simulink model "Channelizer"  (R2023a)
settings: Solver=VariableStepAuto  StartTime=0.0  StopTime=inf  RelTol=1e-3
InitFcn:
  | init;
values from neighbouring files (symbols this model uses):
  ch0_en = 0    [init.m]
  ch0_qam = 0    [init.m]
  ch0_swp = 0    [init.m]
  ch10_en = 0    [init.m]
  ch10_qam = 0    [init.m]
  ch10_swp = 0    [init.m]
  ch11_en = 0    [init.m]
  ch11_qam = 0    [init.m]
  ch11_swp = 0    [init.m]
  ch12_en = 0    [init.m]
  ch12_qam = 0    [init.m]
  ch12_swp = 0    [init.m]
  ch13_en = 0    [init.m]
  ch13_qam = 0    [init.m]
  ch13_swp = 0    [init.m]
  ch14_en = 0    [init.m]
  ch14_qam = 0    [init.m]
  ch14_swp = 0    [init.m]
  ch15_en = 0    [init.m]
  ch15_qam = 0    [init.m]
  ch15_swp = 0    [init.m]
  ch1_en = 1    [init.m]
  ch1_qam = 0    [init.m]
  ch1_swp = 0    [init.m]
  ch2_en = 1    [init.m]
  ch2_qam = 0    [init.m]
  ch2_swp = 0    [init.m]
  ch3_en = 0    [init.m]
  ch3_qam = 0    [init.m]
  ch3_swp = 0    [init.m]
  ch4_en = 0    [init.m]
  ch4_qam = 0    [init.m]
  ch4_swp = 0    [init.m]
  ch5_en = 1    [init.m]
  ch5_qam = 1    [init.m]
  ch5_swp = 0    [init.m]
  ch6_en = 1    [init.m]
  ch6_qam = 1    [init.m]
  ch6_swp = 0    [init.m]
  ch7_en = 0    [init.m]
  ch7_qam = 0    [init.m]
  ch7_swp = 0    [init.m]
  ch8_en = 0    [init.m]
  ch8_qam = 0    [init.m]
  ch8_swp = 0    [init.m]
  ch9_en = 0    [init.m]
  ch9_qam = 0    [init.m]
  ch9_swp = 0    [init.m]
  ch_filt_coef = 28 * ch_filt_coef / sum(ch_filt_coef(:))    [init.m]
  N = 512    [init.m]
  spec1_ch = 1    [init.m]
  spec2_ch = 2    [init.m]
  spec3_ch = 5    [init.m]
  spec4_ch = 6    [init.m]
  swp_rate0 = 0    [init.m]
  swp_rate1 = 0    [init.m]
  swp_rate10 = 0    [init.m]
  swp_rate11 = 0    [init.m]
  swp_rate12 = 0    [init.m]
  swp_rate13 = 0    [init.m]
  swp_rate14 = 0    [init.m]
  swp_rate15 = 0    [init.m]
  swp_rate2 = 0    [init.m]
  swp_rate3 = 0    [init.m]
  swp_rate4 = 0    [init.m]
  swp_rate5 = 0    [init.m]
  swp_rate6 = 0    [init.m]
  swp_rate7 = 0    [init.m]
  swp_rate8 = 0    [init.m]
  swp_rate9 = 0    [init.m]
  Ts = 16*(7/4)/8.75e9    (= 3.2e-09)    [init.m]
undefined symbols (not defined in the file or in its folder): S, vsva2197, xcvc1902
libraries: aieBasic x56, aieUtilities x47, dspswit3 x16, dspsigops x16, hlsBasic x3, dspindex x1, vmcUtilities x1, commchan3 x1
(part 3 of 4)

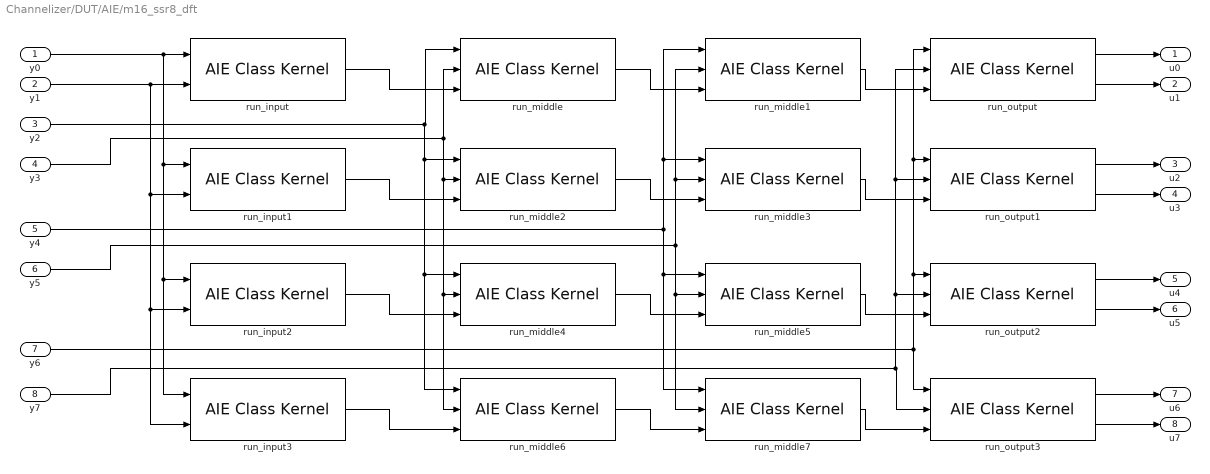
== system Channelizer/DUT/AIE/m16_ssr8_dft ==
  y0 : Inport
  y1 : Inport  Port=2
  y2 : Inport  Port=3
  y3 : Inport  Port=4
  y4 : Inport  Port=5
  y5 : Inport  Port=6
  y6 : Inport  Port=7
  y7 : Inport  Port=8
  run_input : aieBasic/AIE Class Kernel  KernelAllAttrs=|  PortNames={'sig0_i'; 'sig1_i'; 'acc_o'}  PortSerializedTypes={'{Q2{P{Tinput_stream{1{t{ETT_DATA}}}}}}'; '{Q2{P{Tinput_stream{1{t{ETT_DATA}}}}}}'; '{Q2{P{Toutput_stream{1{t{ETT_ACC}}}}}}'}  PortWindowSizes={0.000000000000000000e+00; 0.000000000000000000e+00; 0.000000000000000000e+00}  PortWindowMargins={0.000000000000000000e+00; 0.000000000000000000e+00; 0.000000000000000000e+00}  PortSynchronicities={'auto', 'auto', 'auto'}  PortSignalSizes={0.000000000000000000e+00; 0.000000000000000000e+00; 4.096000000000000000e+03}  ClassTemplateSpecKind=implicit  ClassTemplateParamNames={'TT_DATA'; 'TT_COEFF'; 'TT_ACC'; 'NSAMP'}  ClassTemplateParamKinds={'type'; 'type'; 'type'; 'nontype'}  ClassTemplateParamTypes={'typename'; 'typename'; 'typename'; 'unsigned int'}  ClassTemplateParamValues={'cint16', 'cint16', 'cacc48', '2048'}  ClassCtorParamNames={'coeff0_i'; 'coeff1_i'}  ClassCtorParamSerializedTypes={'{R{C{ETT_COEFF}8}}'; '{R{C{ETT_COEFF}8}}'}  ClassCtorParamValues={'[32767 32767 32767 32767 32767 30274+12540i 23170+23170i 12540+30274i]', '[32767 23170+23170i 0+32767i -23170+23170i 32767 12540+30274i -23170+23170i -30274-12540i]'}  ClassIndex=1  ClassCtorIndex=1  ClassTabVisible=on  ClassTemplateParamsVisible=on  ClassCtorDeclVisible=on  ClassCtorParamsVisible=on  FunctionTabVisible=on  FunctionDecl=|  PortAttrs={ 'input', 'sig0_i', 'input_stream< TT_DATA > * restrict', '', '', '', ''; 'input', 'sig1_i', 'input_stream< TT_DATA > * restrict', '', '', '', ''; 'output', 'acc_o', 'output_stream< TT_ACC > * restrict', '', '', '', '8*N' }  PortAttrsEnables={'off', 'off', 'off', 'off', 'off', 'off', 'off';'off', 'off', 'off', 'off', 'off', 'off', 'off';'off', 'off', 'off', 'off', 'off', 'off', 'on'}  SampleTime=-1  ClassDeclTypeOptions=C[1 1]@t106@template < typename TT_DATA, typename TT_COEFF, typename TT_ACC, unsigned int NSAMP > class dft_1xN_input;  ClassDecl=template < typename TT_DATA, typename TT_COEFF, typename TT_ACC, unsigned int NSAMP > class dft_1xN_input;  ClassTemplateParams={ 'TT_DATA', 'typename', 'cint16'; 'TT_COEFF', 'typename', 'cint16'; 'TT_ACC', 'typename', 'cacc48'; 'NSAMP', 'unsigned int', '4*N' }  ClassTemplateParamsEnables={'off', 'off', 'on';'off', 'off', 'on';'off', 'off', 'on';'off', 'off', 'on'}  ClassCtorDeclTypeOptions=C[1 1]@t75@dft_1xN_input(TT_COEFF ( & coeff0_i ) [ 8 ], TT_COEFF ( & coeff1_i ) [ 8 ])  ClassCtorDecl=dft_1xN_input(TT_COEFF ( & coeff0_i ) [ 8 ], TT_COEFF ( & coeff1_i ) [ 8 ])  ClassCtorParams={ 'coeff0_i', 'TT_COEFF ( &) [ 8 ]', 'twidA0(1,:)'; 'coeff1_i', 'TT_COEFF ( &) [ 8 ]', 'twidA1(1,:)' }  KernelHeaderFile=aie/dft_1xN_widget.h  KernelClassName=dft_1xN_input  KernelFunction=run_input  KernelSourceFile=aie/dft_1xN_widget.cpp  KernelSearchPaths={}  PreProcOptions={}  blockJsonConstraints=[]
      KernelAllAttrs=|
      | s[12;12;9;9;19;14;21;23;21;23;24;21;15;17;12;24;26;26;26;27;28;9;21;23;23;23;24;25;14;19;19;29]@FunctionNameDeclFileNamePortNamesPortTypesPortSerializedTypesPortDirectionsPortWindowSizeEnablesPortWindowMarginEnablesPortBufferSizeEnablesPortBufferMarginEnablesPortSynchronicityEnablesPortSignalSizeEnablesPortBufferSizesPortBufferMarginsFunctionDeclFunctionTemplateSpecKindFunctionTemplateParamNamesFunctionTemplateParamKindsFunctionTemplateParamTypesFunctionTemplateParamValuesFunctionTemplateParamEnablesClassDeclClassTemplateSpecKindClassTemplateParamNamesClassTemplateParamKindsClassTemplateParamTypesClassTemplateParamValuesClassTemplateParamEnablesClassCtorDeclsClassCtorParamNamesClassCtorParamTypesClassCtorParamSerializedTypes[1 1]@C[32 1]@t9@run_inputt22@../../dft_1xN_widget.hC[3 1]@t6@sig0_it6@sig1_it5@acc_oC[3 1]@t34@input_stream< TT_DATA > * restrictt34@input_stream< TT_DATA > * restrictt34@output_stream< TT_ACC > * restrictC[3 1]@t38@{Q2{P{Tinput_stream{1{t{ETT_DATA}}}}}}t38@{Q2{P{Tinput_stream{1{t{ETT_DATA}}}}}}t38@{Q2{P{Toutput_stream{1{t{ETT_ACC}}}}}}C[3 1]@t5@inputt5@inputt6@outputC[3 1]@l0@l0@l0@C[3 1]@l0@l0@l0@C[3 1]@l0@l0@l0@C[3 1]@l0@l0@l0@C[3 1]@l0@l0@l0@C[3 1]@l0@l0@l1@C[3 1]@nnnC[3 1]@nnnt245@template < typename TT_DATA, typename TT_COEFF, typename TT_ACC, unsigned int NSAMP > 
      | void dft_1xN_input::
      | run_input(input_stream< TT_DATA > * restrict sig0_i, input_stream< TT_DATA > * restrict sig1_i, output_stream< TT_ACC > * restrict acc_o)t4@nonee[0 1]@e[0 1]@e[0 1]@e[0 1]@e[0 1]@t106@template < typename TT_DATA, typename TT_COEFF, typename TT_ACC, unsigned int NSAMP > class dft_1xN_input;t8@implicitC[4 1]@t7@TT_DATAt8@TT_COEFFt6@TT_ACCt5@NSAMPC[4 1]@t4@typet4@typet4@typet7@nontypeC[4 1]@t8@typenamet8@typenamet8@typenamet12@unsigned intC[4 1]@nnnnC[4 1]@l1@l1@l1@l1@C[1 1]@t75@dft_1xN_input(TT_COEFF ( & coeff0_i ) [ 8 ], TT_COEFF ( & coeff1_i ) [ 8 ])C[1 1]@C[2 1]@t8@coeff0_it8@coeff1_iC[1 1]@C[2 1]@t19@TT_COEFF ( &) [ 8 ]t19@TT_COEFF ( &) [ 8 ]C[1 1]@C[2 1]@t18@{R{C{ETT_COEFF}8}}t18@{R{C{ETT_COEFF}8}}
      FunctionDecl=|
      | template < typename TT_DATA, typename TT_COEFF, typename TT_ACC, unsigned int NSAMP > 
      | void dft_1xN_input::
      | run_input(input_stream< TT_DATA > * restrict sig0_i, input_stream< TT_DATA > * restrict sig1_i, output_stream< TT_ACC > * restrict acc_o)
  run_input1 : aieBasic/AIE Class Kernel  KernelAllAttrs=|  PortNames={'sig0_i'; 'sig1_i'; 'acc_o'}  PortSerializedTypes={'{Q2{P{Tinput_stream{1{t{ETT_DATA}}}}}}'; '{Q2{P{Tinput_stream{1{t{ETT_DATA}}}}}}'; '{Q2{P{Toutput_stream{1{t{ETT_ACC}}}}}}'}  PortWindowSizes={0.000000000000000000e+00; 0.000000000000000000e+00; 0.000000000000000000e+00}  PortWindowMargins={0.000000000000000000e+00; 0.000000000000000000e+00; 0.000000000000000000e+00}  PortSynchronicities={'auto', 'auto', 'auto'}  PortSignalSizes={0.000000000000000000e+00; 0.000000000000000000e+00; 4.096000000000000000e+03}  ClassTemplateSpecKind=implicit  ClassTemplateParamNames={'TT_DATA'; 'TT_COEFF'; 'TT_ACC'; 'NSAMP'}  ClassTemplateParamKinds={'type'; 'type'; 'type'; 'nontype'}  ClassTemplateParamTypes={'typename'; 'typename'; 'typename'; 'unsigned int'}  ClassTemplateParamValues={'cint16', 'cint16', 'cacc48', '2048'}  ClassCtorParamNames={'coeff0_i'; 'coeff1_i'}  ClassCtorParamSerializedTypes={'{R{C{ETT_COEFF}8}}'; '{R{C{ETT_COEFF}8}}'}  ClassCtorParamValues={'[32767 32767 32767 32767 0+32767i -12540+30274i -23170+23170i -30274+12540i]', '[-32768 -23170-23170i 0-32768i 23170-23170i 0-32768i 30274-12540i 23170+23170i -12540+30274i]'}  ClassIndex=1  ClassCtorIndex=1  ClassTabVisible=on  ClassTemplateParamsVisible=on  ClassCtorDeclVisible=on  ClassCtorParamsVisible=on  FunctionTabVisible=on  FunctionDecl=|  PortAttrs={ 'input', 'sig0_i', 'input_stream< TT_DATA > * restrict', '', '', '', ''; 'input', 'sig1_i', 'input_stream< TT_DATA > * restrict', '', '', '', ''; 'output', 'acc_o', 'output_stream< TT_ACC > * restrict', '', '', '', '8*N' }  PortAttrsEnables={'off', 'off', 'off', 'off', 'off', 'off', 'off';'off', 'off', 'off', 'off', 'off', 'off', 'off';'off', 'off', 'off', 'off', 'off', 'off', 'on'}  SampleTime=-1  ClassDeclTypeOptions=C[1 1]@t106@template < typename TT_DATA, typename TT_COEFF, typename TT_ACC, unsigned int NSAMP > class dft_1xN_input;  ClassDecl=template < typename TT_DATA, typename TT_COEFF, typename TT_ACC, unsigned int NSAMP > class dft_1xN_input;  ClassTemplateParams={ 'TT_DATA', 'typename', 'cint16'; 'TT_COEFF', 'typename', 'cint16'; 'TT_ACC', 'typename', 'cacc48'; 'NSAMP', 'unsigned int', '4*N' }  ClassTemplateParamsEnables={'off', 'off', 'on';'off', 'off', 'on';'off', 'off', 'on';'off', 'off', 'on'}  ClassCtorDeclTypeOptions=C[1 1]@t75@dft_1xN_input(TT_COEFF ( & coeff0_i ) [ 8 ], TT_COEFF ( & coeff1_i ) [ 8 ])  ClassCtorDecl=dft_1xN_input(TT_COEFF ( & coeff0_i ) [ 8 ], TT_COEFF ( & coeff1_i ) [ 8 ])  ClassCtorParams={ 'coeff0_i', 'TT_COEFF ( &) [ 8 ]', 'twidB0(1,:)'; 'coeff1_i', 'TT_COEFF ( &) [ 8 ]', 'twidB1(1,:)' }  KernelHeaderFile=aie/dft_1xN_widget.h  KernelClassName=dft_1xN_input  KernelFunction=run_input  KernelSourceFile=aie/dft_1xN_widget.cpp  KernelSearchPaths={}  PreProcOptions={}  blockJsonConstraints=[]
      KernelAllAttrs=|
      | s[12;12;9;9;19;14;21;23;21;23;24;21;15;17;12;24;26;26;26;27;28;9;21;23;23;23;24;25;14;19;19;29]@FunctionNameDeclFileNamePortNamesPortTypesPortSerializedTypesPortDirectionsPortWindowSizeEnablesPortWindowMarginEnablesPortBufferSizeEnablesPortBufferMarginEnablesPortSynchronicityEnablesPortSignalSizeEnablesPortBufferSizesPortBufferMarginsFunctionDeclFunctionTemplateSpecKindFunctionTemplateParamNamesFunctionTemplateParamKindsFunctionTemplateParamTypesFunctionTemplateParamValuesFunctionTemplateParamEnablesClassDeclClassTemplateSpecKindClassTemplateParamNamesClassTemplateParamKindsClassTemplateParamTypesClassTemplateParamValuesClassTemplateParamEnablesClassCtorDeclsClassCtorParamNamesClassCtorParamTypesClassCtorParamSerializedTypes[1 1]@C[32 1]@t9@run_inputt22@../../dft_1xN_widget.hC[3 1]@t6@sig0_it6@sig1_it5@acc_oC[3 1]@t34@input_stream< TT_DATA > * restrictt34@input_stream< TT_DATA > * restrictt34@output_stream< TT_ACC > * restrictC[3 1]@t38@{Q2{P{Tinput_stream{1{t{ETT_DATA}}}}}}t38@{Q2{P{Tinput_stream{1{t{ETT_DATA}}}}}}t38@{Q2{P{Toutput_stream{1{t{ETT_ACC}}}}}}C[3 1]@t5@inputt5@inputt6@outputC[3 1]@l0@l0@l0@C[3 1]@l0@l0@l0@C[3 1]@l0@l0@l0@C[3 1]@l0@l0@l0@C[3 1]@l0@l0@l0@C[3 1]@l0@l0@l1@C[3 1]@nnnC[3 1]@nnnt245@template < typename TT_DATA, typename TT_COEFF, typename TT_ACC, unsigned int NSAMP > 
      | void dft_1xN_input::
      | run_input(input_stream< TT_DATA > * restrict sig0_i, input_stream< TT_DATA > * restrict sig1_i, output_stream< TT_ACC > * restrict acc_o)t4@nonee[0 1]@e[0 1]@e[0 1]@e[0 1]@e[0 1]@t106@template < typename TT_DATA, typename TT_COEFF, typename TT_ACC, unsigned int NSAMP > class dft_1xN_input;t8@implicitC[4 1]@t7@TT_DATAt8@TT_COEFFt6@TT_ACCt5@NSAMPC[4 1]@t4@typet4@typet4@typet7@nontypeC[4 1]@t8@typenamet8@typenamet8@typenamet12@unsigned intC[4 1]@nnnnC[4 1]@l1@l1@l1@l1@C[1 1]@t75@dft_1xN_input(TT_COEFF ( & coeff0_i ) [ 8 ], TT_COEFF ( & coeff1_i ) [ 8 ])C[1 1]@C[2 1]@t8@coeff0_it8@coeff1_iC[1 1]@C[2 1]@t19@TT_COEFF ( &) [ 8 ]t19@TT_COEFF ( &) [ 8 ]C[1 1]@C[2 1]@t18@{R{C{ETT_COEFF}8}}t18@{R{C{ETT_COEFF}8}}
      FunctionDecl=|
      | template < typename TT_DATA, typename TT_COEFF, typename TT_ACC, unsigned int NSAMP > 
      | void dft_1xN_input::
      | run_input(input_stream< TT_DATA > * restrict sig0_i, input_stream< TT_DATA > * restrict sig1_i, output_stream< TT_ACC > * restrict acc_o)
  run_input2 : aieBasic/AIE Class Kernel  KernelAllAttrs=|  PortNames={'sig0_i'; 'sig1_i'; 'acc_o'}  PortSerializedTypes={'{Q2{P{Tinput_stream{1{t{ETT_DATA}}}}}}'; '{Q2{P{Tinput_stream{1{t{ETT_DATA}}}}}}'; '{Q2{P{Toutput_stream{1{t{ETT_ACC}}}}}}'}  PortWindowSizes={0.000000000000000000e+00; 0.000000000000000000e+00; 0.000000000000000000e+00}  PortWindowMargins={0.000000000000000000e+00; 0.000000000000000000e+00; 0.000000000000000000e+00}  PortSynchronicities={'auto', 'auto', 'auto'}  PortSignalSizes={0.000000000000000000e+00; 0.000000000000000000e+00; 4.096000000000000000e+03}  ClassTemplateSpecKind=implicit  ClassTemplateParamNames={'TT_DATA'; 'TT_COEFF'; 'TT_ACC'; 'NSAMP'}  ClassTemplateParamKinds={'type'; 'type'; 'type'; 'nontype'}  ClassTemplateParamTypes={'typename'; 'typename'; 'typename'; 'unsigned int'}  ClassTemplateParamValues={'cint16', 'cint16', 'cacc48', '2048'}  ClassCtorParamNames={'coeff0_i'; 'coeff1_i'}  ClassCtorParamSerializedTypes={'{R{C{ETT_COEFF}8}}'; '{R{C{ETT_COEFF}8}}'}  ClassCtorParamValues={'[32767 32767 32767 32767 -32768 -30274-12540i -23170-23170i -12540-30274i]', '[32767 23170+23170i 0+32767i -23170+23170i -32768 -12540-30274i 23170-23170i 30274+12540i]'}  ClassIndex=1  ClassCtorIndex=1  ClassTabVisible=on  ClassTemplateParamsVisible=on  ClassCtorDeclVisible=on  ClassCtorParamsVisible=on  FunctionTabVisible=on  FunctionDecl=|  PortAttrs={ 'input', 'sig0_i', 'input_stream< TT_DATA > * restrict', '', '', '', ''; 'input', 'sig1_i', 'input_stream< TT_DATA > * restrict', '', '', '', ''; 'output', 'acc_o', 'output_stream< TT_ACC > * restrict', '', '', '', '8*N' }  PortAttrsEnables={'off', 'off', 'off', 'off', 'off', 'off', 'off';'off', 'off', 'off', 'off', 'off', 'off', 'off';'off', 'off', 'off', 'off', 'off', 'off', 'on'}  SampleTime=-1  ClassDeclTypeOptions=C[1 1]@t106@template < typename TT_DATA, typename TT_COEFF, typename TT_ACC, unsigned int NSAMP > class dft_1xN_input;  ClassDecl=template < typename TT_DATA, typename TT_COEFF, typename TT_ACC, unsigned int NSAMP > class dft_1xN_input;  ClassTemplateParams={ 'TT_DATA', 'typename', 'cint16'; 'TT_COEFF', 'typename', 'cint16'; 'TT_ACC', 'typename', 'cacc48'; 'NSAMP', 'unsigned int', '4*N' }  ClassTemplateParamsEnables={'off', 'off', 'on';'off', 'off', 'on';'off', 'off', 'on';'off', 'off', 'on'}  ClassCtorDeclTypeOptions=C[1 1]@t75@dft_1xN_input(TT_COEFF ( & coeff0_i ) [ 8 ], TT_COEFF ( & coeff1_i ) [ 8 ])  ClassCtorDecl=dft_1xN_input(TT_COEFF ( & coeff0_i ) [ 8 ], TT_COEFF ( & coeff1_i ) [ 8 ])  ClassCtorParams={ 'coeff0_i', 'TT_COEFF ( &) [ 8 ]', 'twidC0(1,:)'; 'coeff1_i', 'TT_COEFF ( &) [ 8 ]', 'twidC1(1,:)' }  KernelHeaderFile=aie/dft_1xN_widget.h  KernelClassName=dft_1xN_input  KernelFunction=run_input  KernelSourceFile=aie/dft_1xN_widget.cpp  KernelSearchPaths={}  PreProcOptions={}  blockJsonConstraints=[]
      KernelAllAttrs=|
      | s[12;12;9;9;19;14;21;23;21;23;24;21;15;17;12;24;26;26;26;27;28;9;21;23;23;23;24;25;14;19;19;29]@FunctionNameDeclFileNamePortNamesPortTypesPortSerializedTypesPortDirectionsPortWindowSizeEnablesPortWindowMarginEnablesPortBufferSizeEnablesPortBufferMarginEnablesPortSynchronicityEnablesPortSignalSizeEnablesPortBufferSizesPortBufferMarginsFunctionDeclFunctionTemplateSpecKindFunctionTemplateParamNamesFunctionTemplateParamKindsFunctionTemplateParamTypesFunctionTemplateParamValuesFunctionTemplateParamEnablesClassDeclClassTemplateSpecKindClassTemplateParamNamesClassTemplateParamKindsClassTemplateParamTypesClassTemplateParamValuesClassTemplateParamEnablesClassCtorDeclsClassCtorParamNamesClassCtorParamTypesClassCtorParamSerializedTypes[1 1]@C[32 1]@t9@run_inputt22@../../dft_1xN_widget.hC[3 1]@t6@sig0_it6@sig1_it5@acc_oC[3 1]@t34@input_stream< TT_DATA > * restrictt34@input_stream< TT_DATA > * restrictt34@output_stream< TT_ACC > * restrictC[3 1]@t38@{Q2{P{Tinput_stream{1{t{ETT_DATA}}}}}}t38@{Q2{P{Tinput_stream{1{t{ETT_DATA}}}}}}t38@{Q2{P{Toutput_stream{1{t{ETT_ACC}}}}}}C[3 1]@t5@inputt5@inputt6@outputC[3 1]@l0@l0@l0@C[3 1]@l0@l0@l0@C[3 1]@l0@l0@l0@C[3 1]@l0@l0@l0@C[3 1]@l0@l0@l0@C[3 1]@l0@l0@l1@C[3 1]@nnnC[3 1]@nnnt245@template < typename TT_DATA, typename TT_COEFF, typename TT_ACC, unsigned int NSAMP > 
      | void dft_1xN_input::
      | run_input(input_stream< TT_DATA > * restrict sig0_i, input_stream< TT_DATA > * restrict sig1_i, output_stream< TT_ACC > * restrict acc_o)t4@nonee[0 1]@e[0 1]@e[0 1]@e[0 1]@e[0 1]@t106@template < typename TT_DATA, typename TT_COEFF, typename TT_ACC, unsigned int NSAMP > class dft_1xN_input;t8@implicitC[4 1]@t7@TT_DATAt8@TT_COEFFt6@TT_ACCt5@NSAMPC[4 1]@t4@typet4@typet4@typet7@nontypeC[4 1]@t8@typenamet8@typenamet8@typenamet12@unsigned intC[4 1]@nnnnC[4 1]@l1@l1@l1@l1@C[1 1]@t75@dft_1xN_input(TT_COEFF ( & coeff0_i ) [ 8 ], TT_COEFF ( & coeff1_i ) [ 8 ])C[1 1]@C[2 1]@t8@coeff0_it8@coeff1_iC[1 1]@C[2 1]@t19@TT_COEFF ( &) [ 8 ]t19@TT_COEFF ( &) [ 8 ]C[1 1]@C[2 1]@t18@{R{C{ETT_COEFF}8}}t18@{R{C{ETT_COEFF}8}}
      FunctionDecl=|
      | template < typename TT_DATA, typename TT_COEFF, typename TT_ACC, unsigned int NSAMP > 
      | void dft_1xN_input::
      | run_input(input_stream< TT_DATA > * restrict sig0_i, input_stream< TT_DATA > * restrict sig1_i, output_stream< TT_ACC > * restrict acc_o)
  run_input3 : aieBasic/AIE Class Kernel  KernelAllAttrs=|  PortNames={'sig0_i'; 'sig1_i'; 'acc_o'}  PortSerializedTypes={'{Q2{P{Tinput_stream{1{t{ETT_DATA}}}}}}'; '{Q2{P{Tinput_stream{1{t{ETT_DATA}}}}}}'; '{Q2{P{Toutput_stream{1{t{ETT_ACC}}}}}}'}  PortWindowSizes={0.000000000000000000e+00; 0.000000000000000000e+00; 0.000000000000000000e+00}  PortWindowMargins={0.000000000000000000e+00; 0.000000000000000000e+00; 0.000000000000000000e+00}  PortSynchronicities={'auto', 'auto', 'auto'}  PortSignalSizes={0.000000000000000000e+00; 0.000000000000000000e+00; 4.096000000000000000e+03}  ClassTemplateSpecKind=implicit  ClassTemplateParamNames={'TT_DATA'; 'TT_COEFF'; 'TT_ACC'; 'NSAMP'}  ClassTemplateParamKinds={'type'; 'type'; 'type'; 'nontype'}  ClassTemplateParamTypes={'typename'; 'typename'; 'typename'; 'unsigned int'}  ClassTemplateParamValues={'cint16', 'cint16', 'cacc48', '2048'}  ClassCtorParamNames={'coeff0_i'; 'coeff1_i'}  ClassCtorParamSerializedTypes={'{R{C{ETT_COEFF}8}}'; '{R{C{ETT_COEFF}8}}'}  ClassCtorParamValues={'[32767 32767 32767 32767 0-32768i 12540-30274i 23170-23170i 30274-12540i]', '[-32768 -23170-23170i 0-32768i 23170-23170i 0+32767i -30274+12540i -23170-23170i 12540-30274i]'}  ClassIndex=1  ClassCtorIndex=1  ClassTabVisible=on  ClassTemplateParamsVisible=on  ClassCtorDeclVisible=on  ClassCtorParamsVisible=on  FunctionTabVisible=on  FunctionDecl=|  PortAttrs={ 'input', 'sig0_i', 'input_stream< TT_DATA > * restrict', '', '', '', ''; 'input', 'sig1_i', 'input_stream< TT_DATA > * restrict', '', '', '', ''; 'output', 'acc_o', 'output_stream< TT_ACC > * restrict', '', '', '', '8*N' }  PortAttrsEnables={'off', 'off', 'off', 'off', 'off', 'off', 'off';'off', 'off', 'off', 'off', 'off', 'off', 'off';'off', 'off', 'off', 'off', 'off', 'off', 'on'}  SampleTime=-1  ClassDeclTypeOptions=C[1 1]@t106@template < typename TT_DATA, typename TT_COEFF, typename TT_ACC, unsigned int NSAMP > class dft_1xN_input;  ClassDecl=template < typename TT_DATA, typename TT_COEFF, typename TT_ACC, unsigned int NSAMP > class dft_1xN_input;  ClassTemplateParams={ 'TT_DATA', 'typename', 'cint16'; 'TT_COEFF', 'typename', 'cint16'; 'TT_ACC', 'typename', 'cacc48'; 'NSAMP', 'unsigned int', '4*N' }  ClassTemplateParamsEnables={'off', 'off', 'on';'off', 'off', 'on';'off', 'off', 'on';'off', 'off', 'on'}  ClassCtorDeclTypeOptions=C[1 1]@t75@dft_1xN_input(TT_COEFF ( & coeff0_i ) [ 8 ], TT_COEFF ( & coeff1_i ) [ 8 ])  ClassCtorDecl=dft_1xN_input(TT_COEFF ( & coeff0_i ) [ 8 ], TT_COEFF ( & coeff1_i ) [ 8 ])  ClassCtorParams={ 'coeff0_i', 'TT_COEFF ( &) [ 8 ]', 'twidD0(1,:)'; 'coeff1_i', 'TT_COEFF ( &) [ 8 ]', 'twidD1(1,:)' }  KernelHeaderFile=aie/dft_1xN_widget.h  KernelClassName=dft_1xN_input  KernelFunction=run_input  KernelSourceFile=aie/dft_1xN_widget.cpp  KernelSearchPaths={}  PreProcOptions={}  blockJsonConstraints=[]
      KernelAllAttrs=|
      | s[12;12;9;9;19;14;21;23;21;23;24;21;15;17;12;24;26;26;26;27;28;9;21;23;23;23;24;25;14;19;19;29]@FunctionNameDeclFileNamePortNamesPortTypesPortSerializedTypesPortDirectionsPortWindowSizeEnablesPortWindowMarginEnablesPortBufferSizeEnablesPortBufferMarginEnablesPortSynchronicityEnablesPortSignalSizeEnablesPortBufferSizesPortBufferMarginsFunctionDeclFunctionTemplateSpecKindFunctionTemplateParamNamesFunctionTemplateParamKindsFunctionTemplateParamTypesFunctionTemplateParamValuesFunctionTemplateParamEnablesClassDeclClassTemplateSpecKindClassTemplateParamNamesClassTemplateParamKindsClassTemplateParamTypesClassTemplateParamValuesClassTemplateParamEnablesClassCtorDeclsClassCtorParamNamesClassCtorParamTypesClassCtorParamSerializedTypes[1 1]@C[32 1]@t9@run_inputt22@../../dft_1xN_widget.hC[3 1]@t6@sig0_it6@sig1_it5@acc_oC[3 1]@t34@input_stream< TT_DATA > * restrictt34@input_stream< TT_DATA > * restrictt34@output_stream< TT_ACC > * restrictC[3 1]@t38@{Q2{P{Tinput_stream{1{t{ETT_DATA}}}}}}t38@{Q2{P{Tinput_stream{1{t{ETT_DATA}}}}}}t38@{Q2{P{Toutput_stream{1{t{ETT_ACC}}}}}}C[3 1]@t5@inputt5@inputt6@outputC[3 1]@l0@l0@l0@C[3 1]@l0@l0@l0@C[3 1]@l0@l0@l0@C[3 1]@l0@l0@l0@C[3 1]@l0@l0@l0@C[3 1]@l0@l0@l1@C[3 1]@nnnC[3 1]@nnnt245@template < typename TT_DATA, typename TT_COEFF, typename TT_ACC, unsigned int NSAMP > 
      | void dft_1xN_input::
      | run_input(input_stream< TT_DATA > * restrict sig0_i, input_stream< TT_DATA > * restrict sig1_i, output_stream< TT_ACC > * restrict acc_o)t4@nonee[0 1]@e[0 1]@e[0 1]@e[0 1]@e[0 1]@t106@template < typename TT_DATA, typename TT_COEFF, typename TT_ACC, unsigned int NSAMP > class dft_1xN_input;t8@implicitC[4 1]@t7@TT_DATAt8@TT_COEFFt6@TT_ACCt5@NSAMPC[4 1]@t4@typet4@typet4@typet7@nontypeC[4 1]@t8@typenamet8@typenamet8@typenamet12@unsigned intC[4 1]@nnnnC[4 1]@l1@l1@l1@l1@C[1 1]@t75@dft_1xN_input(TT_COEFF ( & coeff0_i ) [ 8 ], TT_COEFF ( & coeff1_i ) [ 8 ])C[1 1]@C[2 1]@t8@coeff0_it8@coeff1_iC[1 1]@C[2 1]@t19@TT_COEFF ( &) [ 8 ]t19@TT_COEFF ( &) [ 8 ]C[1 1]@C[2 1]@t18@{R{C{ETT_COEFF}8}}t18@{R{C{ETT_COEFF}8}}
      FunctionDecl=|
      | template < typename TT_DATA, typename TT_COEFF, typename TT_ACC, unsigned int NSAMP > 
      | void dft_1xN_input::
      | run_input(input_stream< TT_DATA > * restrict sig0_i, input_stream< TT_DATA > * restrict sig1_i, output_stream< TT_ACC > * restrict acc_o)
  run_middle : aieBasic/AIE Class Kernel  KernelAllAttrs=|  PortNames={'sig0_i'; 'sig1_i'; 'acc_i'; 'acc_o'}  PortSerializedTypes={'{Q2{P{Tinput_stream{1{t{ETT_DATA}}}}}}'; '{Q2{P{Tinput_stream{1{t{ETT_DATA}}}}}}'; '{Q2{P{Tinput_stream{1{t{ETT_ACC}}}}}}'; '{Q2{P{Toutput_stream{1{t{ETT_ACC}}}}}}'}  PortWindowSizes={0.000000000000000000e+00; 0.000000000000000000e+00; 0.000000000000000000e+00; 0.000000000000000000e+00}  PortWindowMargins={0.000000000000000000e+00; 0.000000000000000000e+00; 0.000000000000000000e+00; 0.000000000000000000e+00}  PortSynchronicities={'auto', 'auto', 'auto', 'auto'}  PortSignalSizes={0.000000000000000000e+00; 0.000000000000000000e+00; 0.000000000000000000e+00; 4.096000000000000000e+03}  ClassTemplateSpecKind=implicit  ClassTemplateParamNames={'TT_DATA'; 'TT_COEFF'; 'TT_ACC'; 'NSAMP'}  ClassTemplateParamKinds={'type'; 'type'; 'type'; 'nontype'}  ClassTemplateParamTypes={'typename'; 'typename'; 'typename'; 'unsigned int'}  ClassTemplateParamValues={'cint16', 'cint16', 'cacc48', '2048'}  ClassCtorParamNames={'coeff0_i'; 'coeff1_i'}  ClassCtorParamSerializedTypes={'{R{C{ETT_COEFF}8}}'; '{R{C{ETT_COEFF}8}}'}  ClassCtorParamValues={'[32767 0+32767i -32768 0-32768i 32767 -12540+30274i -23170-23170i 30274-12540i]', '[32767 -23170+23170i 0-32768i 23170+23170i 32767 -30274+12540i 23170-23170i -12540+30274i]'}  ClassIndex=1  ClassCtorIndex=1  ClassTabVisible=on  ClassTemplateParamsVisible=on  ClassCtorDeclVisible=on  ClassCtorParamsVisible=on  FunctionTabVisible=on  FunctionDecl=|  PortAttrs={ 'input', 'sig0_i', 'input_stream< TT_DATA > * restrict', '', '', '', ''; 'input', 'sig1_i', 'input_stream< TT_DATA > * restrict', '', '', '', ''; 'input', 'acc_i', 'input_stream< TT_ACC > * restrict', '', '', '', ''; 'output', 'acc_o', 'output_stream< TT_ACC > * restrict', '', '', '', '8*N' }  PortAttrsEnables={'off', 'off', 'off', 'off', 'off', 'off', 'off';'off', 'off', 'off', 'off', 'off', 'off', 'off';'off', 'off', 'off', 'off', 'off', 'off', 'off';'off', 'off', 'off', 'off', 'off', 'off', 'on'}  SampleTime=-1  ClassDeclTypeOptions=C[1 1]@t107@template < typename TT_DATA, typename TT_COEFF, typename TT_ACC, unsigned int NSAMP > class dft_1xN_middle;  ClassDecl=template < typename TT_DATA, typename TT_COEFF, typename TT_ACC, unsigned int NSAMP > class dft_1xN_middle;  ClassTemplateParams={ 'TT_DATA', 'typename', 'cint16'; 'TT_COEFF', 'typename', 'cint16'; 'TT_ACC', 'typename', 'cacc48'; 'NSAMP', 'unsigned int', '4*N' }  ClassTemplateParamsEnables={'off', 'off', 'on';'off', 'off', 'on';'off', 'off', 'on';'off', 'off', 'on'}  ClassCtorDeclTypeOptions=C[1 1]@t76@dft_1xN_middle(TT_COEFF ( & coeff0_i ) [ 8 ], TT_COEFF ( & coeff1_i ) [ 8 ])  ClassCtorDecl=dft_1xN_middle(TT_COEFF ( & coeff0_i ) [ 8 ], TT_COEFF ( & coeff1_i ) [ 8 ])  ClassCtorParams={ 'coeff0_i', 'TT_COEFF ( &) [ 8 ]', 'twidA0(2,:)'; 'coeff1_i', 'TT_COEFF ( &) [ 8 ]', 'twidA1(2,:)' }  KernelHeaderFile=aie/dft_1xN_widget.h  KernelClassName=dft_1xN_middle  KernelFunction=run_middle  KernelSourceFile=aie/dft_1xN_widget.cpp  KernelSearchPaths={}  PreProcOptions={}  blockJsonConstraints=[]
      KernelAllAttrs=|
      | s[12;12;9;9;19;14;21;23;21;23;24;21;15;17;12;24;26;26;26;27;28;9;21;23;23;23;24;25;14;19;19;29]@FunctionNameDeclFileNamePortNamesPortTypesPortSerializedTypesPortDirectionsPortWindowSizeEnablesPortWindowMarginEnablesPortBufferSizeEnablesPortBufferMarginEnablesPortSynchronicityEnablesPortSignalSizeEnablesPortBufferSizesPortBufferMarginsFunctionDeclFunctionTemplateSpecKindFunctionTemplateParamNamesFunctionTemplateParamKindsFunctionTemplateParamTypesFunctionTemplateParamValuesFunctionTemplateParamEnablesClassDeclClassTemplateSpecKindClassTemplateParamNamesClassTemplateParamKindsClassTemplateParamTypesClassTemplateParamValuesClassTemplateParamEnablesClassCtorDeclsClassCtorParamNamesClassCtorParamTypesClassCtorParamSerializedTypes[1 1]@C[32 1]@t10@run_middlet22@../../dft_1xN_widget.hC[4 1]@t6@sig0_it6@sig1_it5@acc_it5@acc_oC[4 1]@t34@input_stream< TT_DATA > * restrictt34@input_stream< TT_DATA > * restrictt33@input_stream< TT_ACC > * restrictt34@output_stream< TT_ACC > * restrictC[4 1]@t38@{Q2{P{Tinput_stream{1{t{ETT_DATA}}}}}}t38@{Q2{P{Tinput_stream{1{t{ETT_DATA}}}}}}t37@{Q2{P{Tinput_stream{1{t{ETT_ACC}}}}}}t38@{Q2{P{Toutput_stream{1{t{ETT_ACC}}}}}}C[4 1]@t5@inputt5@inputt5@inputt6@outputC[4 1]@l0@l0@l0@l0@C[4 1]@l0@l0@l0@l0@C[4 1]@l0@l0@l0@l0@C[4 1]@l0@l0@l0@l0@C[4 1]@l0@l0@l0@l0@C[4 1]@l0@l0@l0@l1@C[4 1]@nnnnC[4 1]@nnnnt288@template < typename TT_DATA, typename TT_COEFF, typename TT_ACC, unsigned int NSAMP > 
      | void dft_1xN_middle::
      | run_middle(input_stream< TT_DATA > * restrict sig0_i, input_stream< TT_DATA > * restrict sig1_i, input_stream< TT_ACC > * restrict acc_i, output_stream< TT_ACC > * restrict acc_o)t4@nonee[0 1]@e[0 1]@e[0 1]@e[0 1]@e[0 1]@t107@template < typename TT_DATA, typename TT_COEFF, typename TT_ACC, unsigned int NSAMP > class dft_1xN_middle;t8@implicitC[4 1]@t7@TT_DATAt8@TT_COEFFt6@TT_ACCt5@NSAMPC[4 1]@t4@typet4@typet4@typet7@nontypeC[4 1]@t8@typenamet8@typenamet8@typenamet12@unsigned intC[4 1]@nnnnC[4 1]@l1@l1@l1@l1@C[1 1]@t76@dft_1xN_middle(TT_COEFF ( & coeff0_i ) [ 8 ], TT_COEFF ( & coeff1_i ) [ 8 ])C[1 1]@C[2 1]@t8@coeff0_it8@coeff1_iC[1 1]@C[2 1]@t19@TT_COEFF ( &) [ 8 ]t19@TT_COEFF ( &) [ 8 ]C[1 1]@C[2 1]@t18@{R{C{ETT_COEFF}8}}t18@{R{C{ETT_COEFF}8}}
      FunctionDecl=|
      | template < typename TT_DATA, typename TT_COEFF, typename TT_ACC, unsigned int NSAMP > 
      | void dft_1xN_middle::
      | run_middle(input_stream< TT_DATA > * restrict sig0_i, input_stream< TT_DATA > * restrict sig1_i, input_stream< TT_ACC > * restrict acc_i, output_stream< TT_ACC > * restrict acc_o)
  run_middle1 : aieBasic/AIE Class Kernel  KernelAllAttrs=|  PortNames={'sig0_i'; 'sig1_i'; 'acc_i'; 'acc_o'}  PortSerializedTypes={'{Q2{P{Tinput_stream{1{t{ETT_DATA}}}}}}'; '{Q2{P{Tinput_stream{1{t{ETT_DATA}}}}}}'; '{Q2{P{Tinput_stream{1{t{ETT_ACC}}}}}}'; '{Q2{P{Toutput_stream{1{t{ETT_ACC}}}}}}'}  PortWindowSizes={0.000000000000000000e+00; 0.000000000000000000e+00; 0.000000000000000000e+00; 0.000000000000000000e+00}  PortWindowMargins={0.000000000000000000e+00; 0.000000000000000000e+00; 0.000000000000000000e+00; 0.000000000000000000e+00}  PortSynchronicities={'auto', 'auto', 'auto', 'auto'}  PortSignalSizes={0.000000000000000000e+00; 0.000000000000000000e+00; 0.000000000000000000e+00; 4.096000000000000000e+03}  ClassTemplateSpecKind=implicit  ClassTemplateParamNames={'TT_DATA'; 'TT_COEFF'; 'TT_ACC'; 'NSAMP'}  ClassTemplateParamKinds={'type'; 'type'; 'type'; 'nontype'}  ClassTemplateParamTypes={'typename'; 'typename'; 'typename'; 'unsigned int'}  ClassTemplateParamValues={'cint16', 'cint16', 'cacc48', '2048'}  ClassCtorParamNames={'coeff0_i'; 'coeff1_i'}  ClassCtorParamSerializedTypes={'{R{C{ETT_COEFF}8}}'; '{R{C{ETT_COEFF}8}}'}  ClassCtorParamValues={'[32767 -32768 32767 -32768 32767 -30274-12540i 23170+23170i -12540-30274i]', '[32767 -23170-23170i 0+32767i 23170-23170i 32767 -12540-30274i -23170+23170i 30274+12540i]'}  ClassIndex=1  ClassCtorIndex=1  ClassTabVisible=on  ClassTemplateParamsVisible=on  ClassCtorDeclVisible=on  ClassCtorParamsVisible=on  FunctionTabVisible=on  FunctionDecl=|  PortAttrs={ 'input', 'sig0_i', 'input_stream< TT_DATA > * restrict', '', '', '', ''; 'input', 'sig1_i', 'input_stream< TT_DATA > * restrict', '', '', '', ''; 'input', 'acc_i', 'input_stream< TT_ACC > * restrict', '', '', '', ''; 'output', 'acc_o', 'output_stream< TT_ACC > * restrict', '', '', '', '8*N' }  PortAttrsEnables={'off', 'off', 'off', 'off', 'off', 'off', 'off';'off', 'off', 'off', 'off', 'off', 'off', 'off';'off', 'off', 'off', 'off', 'off', 'off', 'off';'off', 'off', 'off', 'off', 'off', 'off', 'on'}  SampleTime=-1  ClassDeclTypeOptions=C[1 1]@t107@template < typename TT_DATA, typename TT_COEFF, typename TT_ACC, unsigned int NSAMP > class dft_1xN_middle;  ClassDecl=template < typename TT_DATA, typename TT_COEFF, typename TT_ACC, unsigned int NSAMP > class dft_1xN_middle;  ClassTemplateParams={ 'TT_DATA', 'typename', 'cint16'; 'TT_COEFF', 'typename', 'cint16'; 'TT_ACC', 'typename', 'cacc48'; 'NSAMP', 'unsigned int', '4*N' }  ClassTemplateParamsEnables={'off', 'off', 'on';'off', 'off', 'on';'off', 'off', 'on';'off', 'off', 'on'}  ClassCtorDeclTypeOptions=C[1 1]@t76@dft_1xN_middle(TT_COEFF ( & coeff0_i ) [ 8 ], TT_COEFF ( & coeff1_i ) [ 8 ])  ClassCtorDecl=dft_1xN_middle(TT_COEFF ( & coeff0_i ) [ 8 ], TT_COEFF ( & coeff1_i ) [ 8 ])  ClassCtorParams={ 'coeff0_i', 'TT_COEFF ( &) [ 8 ]', 'twidA0(3,:)'; 'coeff1_i', 'TT_COEFF ( &) [ 8 ]', 'twidA1(3,:)' }  KernelHeaderFile=aie/dft_1xN_widget.h  KernelClassName=dft_1xN_middle  KernelFunction=run_middle  KernelSourceFile=aie/dft_1xN_widget.cpp  KernelSearchPaths={}  PreProcOptions={}  blockJsonConstraints=[]
      KernelAllAttrs=|
      | s[12;12;9;9;19;14;21;23;21;23;24;21;15;17;12;24;26;26;26;27;28;9;21;23;23;23;24;25;14;19;19;29]@FunctionNameDeclFileNamePortNamesPortTypesPortSerializedTypesPortDirectionsPortWindowSizeEnablesPortWindowMarginEnablesPortBufferSizeEnablesPortBufferMarginEnablesPortSynchronicityEnablesPortSignalSizeEnablesPortBufferSizesPortBufferMarginsFunctionDeclFunctionTemplateSpecKindFunctionTemplateParamNamesFunctionTemplateParamKindsFunctionTemplateParamTypesFunctionTemplateParamValuesFunctionTemplateParamEnablesClassDeclClassTemplateSpecKindClassTemplateParamNamesClassTemplateParamKindsClassTemplateParamTypesClassTemplateParamValuesClassTemplateParamEnablesClassCtorDeclsClassCtorParamNamesClassCtorParamTypesClassCtorParamSerializedTypes[1 1]@C[32 1]@t10@run_middlet22@../../dft_1xN_widget.hC[4 1]@t6@sig0_it6@sig1_it5@acc_it5@acc_oC[4 1]@t34@input_stream< TT_DATA > * restrictt34@input_stream< TT_DATA > * restrictt33@input_stream< TT_ACC > * restrictt34@output_stream< TT_ACC > * restrictC[4 1]@t38@{Q2{P{Tinput_stream{1{t{ETT_DATA}}}}}}t38@{Q2{P{Tinput_stream{1{t{ETT_DATA}}}}}}t37@{Q2{P{Tinput_stream{1{t{ETT_ACC}}}}}}t38@{Q2{P{Toutput_stream{1{t{ETT_ACC}}}}}}C[4 1]@t5@inputt5@inputt5@inputt6@outputC[4 1]@l0@l0@l0@l0@C[4 1]@l0@l0@l0@l0@C[4 1]@l0@l0@l0@l0@C[4 1]@l0@l0@l0@l0@C[4 1]@l0@l0@l0@l0@C[4 1]@l0@l0@l0@l1@C[4 1]@nnnnC[4 1]@nnnnt288@template < typename TT_DATA, typename TT_COEFF, typename TT_ACC, unsigned int NSAMP > 
      | void dft_1xN_middle::
      | run_middle(input_stream< TT_DATA > * restrict sig0_i, input_stream< TT_DATA > * restrict sig1_i, input_stream< TT_ACC > * restrict acc_i, output_stream< TT_ACC > * restrict acc_o)t4@nonee[0 1]@e[0 1]@e[0 1]@e[0 1]@e[0 1]@t107@template < typename TT_DATA, typename TT_COEFF, typename TT_ACC, unsigned int NSAMP > class dft_1xN_middle;t8@implicitC[4 1]@t7@TT_DATAt8@TT_COEFFt6@TT_ACCt5@NSAMPC[4 1]@t4@typet4@typet4@typet7@nontypeC[4 1]@t8@typenamet8@typenamet8@typenamet12@unsigned intC[4 1]@nnnnC[4 1]@l1@l1@l1@l1@C[1 1]@t76@dft_1xN_middle(TT_COEFF ( & coeff0_i ) [ 8 ], TT_COEFF ( & coeff1_i ) [ 8 ])C[1 1]@C[2 1]@t8@coeff0_it8@coeff1_iC[1 1]@C[2 1]@t19@TT_COEFF ( &) [ 8 ]t19@TT_COEFF ( &) [ 8 ]C[1 1]@C[2 1]@t18@{R{C{ETT_COEFF}8}}t18@{R{C{ETT_COEFF}8}}
      FunctionDecl=|
      | template < typename TT_DATA, typename TT_COEFF, typename TT_ACC, unsigned int NSAMP > 
      | void dft_1xN_middle::
      | run_middle(input_stream< TT_DATA > * restrict sig0_i, input_stream< TT_DATA > * restrict sig1_i, input_stream< TT_ACC > * restrict acc_i, output_stream< TT_ACC > * restrict acc_o)
  run_middle2 : aieBasic/AIE Class Kernel  KernelAllAttrs=|  PortNames={'sig0_i'; 'sig1_i'; 'acc_i'; 'acc_o'}  PortSerializedTypes={'{Q2{P{Tinput_stream{1{t{ETT_DATA}}}}}}'; '{Q2{P{Tinput_stream{1{t{ETT_DATA}}}}}}'; '{Q2{P{Tinput_stream{1{t{ETT_ACC}}}}}}'; '{Q2{P{Toutput_stream{1{t{ETT_ACC}}}}}}'}  PortWindowSizes={0.000000000000000000e+00; 0.000000000000000000e+00; 0.000000000000000000e+00; 0.000000000000000000e+00}  PortWindowMargins={0.000000000000000000e+00; 0.000000000000000000e+00; 0.000000000000000000e+00; 0.000000000000000000e+00}  PortSynchronicities={'auto', 'auto', 'auto', 'auto'}  PortSignalSizes={0.000000000000000000e+00; 0.000000000000000000e+00; 0.000000000000000000e+00; 4.096000000000000000e+03}  ClassTemplateSpecKind=implicit  ClassTemplateParamNames={'TT_DATA'; 'TT_COEFF'; 'TT_ACC'; 'NSAMP'}  ClassTemplateParamKinds={'type'; 'type'; 'type'; 'nontype'}  ClassTemplateParamTypes={'typename'; 'typename'; 'typename'; 'unsigned int'}  ClassTemplateParamValues={'cint16', 'cint16', 'cacc48', '2048'}  ClassCtorParamNames={'coeff0_i'; 'coeff1_i'}  ClassCtorParamSerializedTypes={'{R{C{ETT_COEFF}8}}'; '{R{C{ETT_COEFF}8}}'}  ClassCtorParamValues={'[32767 0+32767i -32768 0-32768i 0+32767i -30274-12540i 23170-23170i 12540+30274i]', '[-32768 23170-23170i 0+32767i -23170-23170i 0-32768i 12540+30274i -23170-23170i 30274+12540i]'}  ClassIndex=1  ClassCtorIndex=1  ClassTabVisible=on  ClassTemplateParamsVisible=on  ClassCtorDeclVisible=on  ClassCtorParamsVisible=on  FunctionTabVisible=on  FunctionDecl=|  PortAttrs={ 'input', 'sig0_i', 'input_stream< TT_DATA > * restrict', '', '', '', ''; 'input', 'sig1_i', 'input_stream< TT_DATA > * restrict', '', '', '', ''; 'input', 'acc_i', 'input_stream< TT_ACC > * restrict', '', '', '', ''; 'output', 'acc_o', 'output_stream< TT_ACC > * restrict', '', '', '', '8*N' }  PortAttrsEnables={'off', 'off', 'off', 'off', 'off', 'off', 'off';'off', 'off', 'off', 'off', 'off', 'off', 'off';'off', 'off', 'off', 'off', 'off', 'off', 'off';'off', 'off', 'off', 'off', 'off', 'off', 'on'}  SampleTime=-1  ClassDeclTypeOptions=C[1 1]@t107@template < typename TT_DATA, typename TT_COEFF, typename TT_ACC, unsigned int NSAMP > class dft_1xN_middle;  ClassDecl=template < typename TT_DATA, typename TT_COEFF, typename TT_ACC, unsigned int NSAMP > class dft_1xN_middle;  ClassTemplateParams={ 'TT_DATA', 'typename', 'cint16'; 'TT_COEFF', 'typename', 'cint16'; 'TT_ACC', 'typename', 'cacc48'; 'NSAMP', 'unsigned int', '4*N' }  ClassTemplateParamsEnables={'off', 'off', 'on';'off', 'off', 'on';'off', 'off', 'on';'off', 'off', 'on'}  ClassCtorDeclTypeOptions=C[1 1]@t76@dft_1xN_middle(TT_COEFF ( & coeff0_i ) [ 8 ], TT_COEFF ( & coeff1_i ) [ 8 ])  ClassCtorDecl=dft_1xN_middle(TT_COEFF ( & coeff0_i ) [ 8 ], TT_COEFF ( & coeff1_i ) [ 8 ])  ClassCtorParams={ 'coeff0_i', 'TT_COEFF ( &) [ 8 ]', 'twidB0(2,:)'; 'coeff1_i', 'TT_COEFF ( &) [ 8 ]', 'twidB1(2,:)' }  KernelHeaderFile=aie/dft_1xN_widget.h  KernelClassName=dft_1xN_middle  KernelFunction=run_middle  KernelSourceFile=aie/dft_1xN_widget.cpp  KernelSearchPaths={}  PreProcOptions={}  blockJsonConstraints=[]
      KernelAllAttrs=|
      | s[12;12;9;9;19;14;21;23;21;23;24;21;15;17;12;24;26;26;26;27;28;9;21;23;23;23;24;25;14;19;19;29]@FunctionNameDeclFileNamePortNamesPortTypesPortSerializedTypesPortDirectionsPortWindowSizeEnablesPortWindowMarginEnablesPortBufferSizeEnablesPortBufferMarginEnablesPortSynchronicityEnablesPortSignalSizeEnablesPortBufferSizesPortBufferMarginsFunctionDeclFunctionTemplateSpecKindFunctionTemplateParamNamesFunctionTemplateParamKindsFunctionTemplateParamTypesFunctionTemplateParamValuesFunctionTemplateParamEnablesClassDeclClassTemplateSpecKindClassTemplateParamNamesClassTemplateParamKindsClassTemplateParamTypesClassTemplateParamValuesClassTemplateParamEnablesClassCtorDeclsClassCtorParamNamesClassCtorParamTypesClassCtorParamSerializedTypes[1 1]@C[32 1]@t10@run_middlet22@../../dft_1xN_widget.hC[4 1]@t6@sig0_it6@sig1_it5@acc_it5@acc_oC[4 1]@t34@input_stream< TT_DATA > * restrictt34@input_stream< TT_DATA > * restrictt33@input_stream< TT_ACC > * restrictt34@output_stream< TT_ACC > * restrictC[4 1]@t38@{Q2{P{Tinput_stream{1{t{ETT_DATA}}}}}}t38@{Q2{P{Tinput_stream{1{t{ETT_DATA}}}}}}t37@{Q2{P{Tinput_stream{1{t{ETT_ACC}}}}}}t38@{Q2{P{Toutput_stream{1{t{ETT_ACC}}}}}}C[4 1]@t5@inputt5@inputt5@inputt6@outputC[4 1]@l0@l0@l0@l0@C[4 1]@l0@l0@l0@l0@C[4 1]@l0@l0@l0@l0@C[4 1]@l0@l0@l0@l0@C[4 1]@l0@l0@l0@l0@C[4 1]@l0@l0@l0@l1@C[4 1]@nnnnC[4 1]@nnnnt288@template < typename TT_DATA, typename TT_COEFF, typename TT_ACC, unsigned int NSAMP > 
      | void dft_1xN_middle::
      | run_middle(input_stream< TT_DATA > * restrict sig0_i, input_stream< TT_DATA > * restrict sig1_i, input_stream< TT_ACC > * restrict acc_i, output_stream< TT_ACC > * restrict acc_o)t4@nonee[0 1]@e[0 1]@e[0 1]@e[0 1]@e[0 1]@t107@template < typename TT_DATA, typename TT_COEFF, typename TT_ACC, unsigned int NSAMP > class dft_1xN_middle;t8@implicitC[4 1]@t7@TT_DATAt8@TT_COEFFt6@TT_ACCt5@NSAMPC[4 1]@t4@typet4@typet4@typet7@nontypeC[4 1]@t8@typenamet8@typenamet8@typenamet12@unsigned intC[4 1]@nnnnC[4 1]@l1@l1@l1@l1@C[1 1]@t76@dft_1xN_middle(TT_COEFF ( & coeff0_i ) [ 8 ], TT_COEFF ( & coeff1_i ) [ 8 ])C[1 1]@C[2 1]@t8@coeff0_it8@coeff1_iC[1 1]@C[2 1]@t19@TT_COEFF ( &) [ 8 ]t19@TT_COEFF ( &) [ 8 ]C[1 1]@C[2 1]@t18@{R{C{ETT_COEFF}8}}t18@{R{C{ETT_COEFF}8}}
      FunctionDecl=|
      | template < typename TT_DATA, typename TT_COEFF, typename TT_ACC, unsigned int NSAMP > 
      | void dft_1xN_middle::
      | run_middle(input_stream< TT_DATA > * restrict sig0_i, input_stream< TT_DATA > * restrict sig1_i, input_stream< TT_ACC > * restrict acc_i, output_stream< TT_ACC > * restrict acc_o)
  run_middle3 : aieBasic/AIE Class Kernel  KernelAllAttrs=|  PortNames={'sig0_i'; 'sig1_i'; 'acc_i'; 'acc_o'}  PortSerializedTypes={'{Q2{P{Tinput_stream{1{t{ETT_DATA}}}}}}'; '{Q2{P{Tinput_stream{1{t{ETT_DATA}}}}}}'; '{Q2{P{Tinput_stream{1{t{ETT_ACC}}}}}}'; '{Q2{P{Toutput_stream{1{t{ETT_ACC}}}}}}'}  PortWindowSizes={0.000000000000000000e+00; 0.000000000000000000e+00; 0.000000000000000000e+00; 0.000000000000000000e+00}  PortWindowMargins={0.000000000000000000e+00; 0.000000000000000000e+00; 0.000000000000000000e+00; 0.000000000000000000e+00}  PortSynchronicities={'auto', 'auto', 'auto', 'auto'}  PortSignalSizes={0.000000000000000000e+00; 0.000000000000000000e+00; 0.000000000000000000e+00; 4.096000000000000000e+03}  ClassTemplateSpecKind=implicit  ClassTemplateParamNames={'TT_DATA'; 'TT_COEFF'; 'TT_ACC'; 'NSAMP'}  ClassTemplateParamKinds={'type'; 'type'; 'type'; 'nontype'}  ClassTemplateParamTypes={'typename'; 'typename'; 'typename'; 'unsigned int'}  ClassTemplateParamValues={'cint16', 'cint16', 'cacc48', '2048'}  ClassCtorParamNames={'coeff0_i'; 'coeff1_i'}  ClassCtorParamSerializedTypes={'{R{C{ETT_COEFF}8}}'; '{R{C{ETT_COEFF}8}}'}  ClassCtorParamValues={'[32767 -32768 32767 -32768 0+32767i 12540-30274i -23170+23170i 30274-12540i]', '[-32768 23170+23170i 0-32768i -23170+23170i 0-32768i -30274+12540i 23170+23170i 12540-30274i]'}  ClassIndex=1  ClassCtorIndex=1  ClassTabVisible=on  ClassTemplateParamsVisible=on  ClassCtorDeclVisible=on  ClassCtorParamsVisible=on  FunctionTabVisible=on  FunctionDecl=|  PortAttrs={ 'input', 'sig0_i', 'input_stream< TT_DATA > * restrict', '', '', '', ''; 'input', 'sig1_i', 'input_stream< TT_DATA > * restrict', '', '', '', ''; 'input', 'acc_i', 'input_stream< TT_ACC > * restrict', '', '', '', ''; 'output', 'acc_o', 'output_stream< TT_ACC > * restrict', '', '', '', '8*N' }  PortAttrsEnables={'off', 'off', 'off', 'off', 'off', 'off', 'off';'off', 'off', 'off', 'off', 'off', 'off', 'off';'off', 'off', 'off', 'off', 'off', 'off', 'off';'off', 'off', 'off', 'off', 'off', 'off', 'on'}  SampleTime=-1  ClassDeclTypeOptions=C[1 1]@t107@template < typename TT_DATA, typename TT_COEFF, typename TT_ACC, unsigned int NSAMP > class dft_1xN_middle;  ClassDecl=template < typename TT_DATA, typename TT_COEFF, typename TT_ACC, unsigned int NSAMP > class dft_1xN_middle;  ClassTemplateParams={ 'TT_DATA', 'typename', 'cint16'; 'TT_COEFF', 'typename', 'cint16'; 'TT_ACC', 'typename', 'cacc48'; 'NSAMP', 'unsigned int', '4*N' }  ClassTemplateParamsEnables={'off', 'off', 'on';'off', 'off', 'on';'off', 'off', 'on';'off', 'off', 'on'}  ClassCtorDeclTypeOptions=C[1 1]@t76@dft_1xN_middle(TT_COEFF ( & coeff0_i ) [ 8 ], TT_COEFF ( & coeff1_i ) [ 8 ])  ClassCtorDecl=dft_1xN_middle(TT_COEFF ( & coeff0_i ) [ 8 ], TT_COEFF ( & coeff1_i ) [ 8 ])  ClassCtorParams={ 'coeff0_i', 'TT_COEFF ( &) [ 8 ]', 'twidB0(3,:)'; 'coeff1_i', 'TT_COEFF ( &) [ 8 ]', 'twidB1(3,:)' }  KernelHeaderFile=aie/dft_1xN_widget.h  KernelClassName=dft_1xN_middle  KernelFunction=run_middle  KernelSourceFile=aie/dft_1xN_widget.cpp  KernelSearchPaths={}  PreProcOptions={}  blockJsonConstraints=[]
      KernelAllAttrs=|
      | s[12;12;9;9;19;14;21;23;21;23;24;21;15;17;12;24;26;26;26;27;28;9;21;23;23;23;24;25;14;19;19;29]@FunctionNameDeclFileNamePortNamesPortTypesPortSerializedTypesPortDirectionsPortWindowSizeEnablesPortWindowMarginEnablesPortBufferSizeEnablesPortBufferMarginEnablesPortSynchronicityEnablesPortSignalSizeEnablesPortBufferSizesPortBufferMarginsFunctionDeclFunctionTemplateSpecKindFunctionTemplateParamNamesFunctionTemplateParamKindsFunctionTemplateParamTypesFunctionTemplateParamValuesFunctionTemplateParamEnablesClassDeclClassTemplateSpecKindClassTemplateParamNamesClassTemplateParamKindsClassTemplateParamTypesClassTemplateParamValuesClassTemplateParamEnablesClassCtorDeclsClassCtorParamNamesClassCtorParamTypesClassCtorParamSerializedTypes[1 1]@C[32 1]@t10@run_middlet22@../../dft_1xN_widget.hC[4 1]@t6@sig0_it6@sig1_it5@acc_it5@acc_oC[4 1]@t34@input_stream< TT_DATA > * restrictt34@input_stream< TT_DATA > * restrictt33@input_stream< TT_ACC > * restrictt34@output_stream< TT_ACC > * restrictC[4 1]@t38@{Q2{P{Tinput_stream{1{t{ETT_DATA}}}}}}t38@{Q2{P{Tinput_stream{1{t{ETT_DATA}}}}}}t37@{Q2{P{Tinput_stream{1{t{ETT_ACC}}}}}}t38@{Q2{P{Toutput_stream{1{t{ETT_ACC}}}}}}C[4 1]@t5@inputt5@inputt5@inputt6@outputC[4 1]@l0@l0@l0@l0@C[4 1]@l0@l0@l0@l0@C[4 1]@l0@l0@l0@l0@C[4 1]@l0@l0@l0@l0@C[4 1]@l0@l0@l0@l0@C[4 1]@l0@l0@l0@l1@C[4 1]@nnnnC[4 1]@nnnnt288@template < typename TT_DATA, typename TT_COEFF, typename TT_ACC, unsigned int NSAMP > 
      | void dft_1xN_middle::
      | run_middle(input_stream< TT_DATA > * restrict sig0_i, input_stream< TT_DATA > * restrict sig1_i, input_stream< TT_ACC > * restrict acc_i, output_stream< TT_ACC > * restrict acc_o)t4@nonee[0 1]@e[0 1]@e[0 1]@e[0 1]@e[0 1]@t107@template < typename TT_DATA, typename TT_COEFF, typename TT_ACC, unsigned int NSAMP > class dft_1xN_middle;t8@implicitC[4 1]@t7@TT_DATAt8@TT_COEFFt6@TT_ACCt5@NSAMPC[4 1]@t4@typet4@typet4@typet7@nontypeC[4 1]@t8@typenamet8@typenamet8@typenamet12@unsigned intC[4 1]@nnnnC[4 1]@l1@l1@l1@l1@C[1 1]@t76@dft_1xN_middle(TT_COEFF ( & coeff0_i ) [ 8 ], TT_COEFF ( & coeff1_i ) [ 8 ])C[1 1]@C[2 1]@t8@coeff0_it8@coeff1_iC[1 1]@C[2 1]@t19@TT_COEFF ( &) [ 8 ]t19@TT_COEFF ( &) [ 8 ]C[1 1]@C[2 1]@t18@{R{C{ETT_COEFF}8}}t18@{R{C{ETT_COEFF}8}}
      FunctionDecl=|
      | template < typename TT_DATA, typename TT_COEFF, typename TT_ACC, unsigned int NSAMP > 
      | void dft_1xN_middle::
      | run_middle(input_stream< TT_DATA > * restrict sig0_i, input_stream< TT_DATA > * restrict sig1_i, input_stream< TT_ACC > * restrict acc_i, output_stream< TT_ACC > * restrict acc_o)
  run_middle4 : aieBasic/AIE Class Kernel  KernelAllAttrs=|  PortNames={'sig0_i'; 'sig1_i'; 'acc_i'; 'acc_o'}  PortSerializedTypes={'{Q2{P{Tinput_stream{1{t{ETT_DATA}}}}}}'; '{Q2{P{Tinput_stream{1{t{ETT_DATA}}}}}}'; '{Q2{P{Tinput_stream{1{t{ETT_ACC}}}}}}'; '{Q2{P{Toutput_stream{1{t{ETT_ACC}}}}}}'}  PortWindowSizes={0.000000000000000000e+00; 0.000000000000000000e+00; 0.000000000000000000e+00; 0.000000000000000000e+00}  PortWindowMargins={0.000000000000000000e+00; 0.000000000000000000e+00; 0.000000000000000000e+00; 0.000000000000000000e+00}  PortSynchronicities={'auto', 'auto', 'auto', 'auto'}  PortSignalSizes={0.000000000000000000e+00; 0.000000000000000000e+00; 0.000000000000000000e+00; 4.096000000000000000e+03}  ClassTemplateSpecKind=implicit  ClassTemplateParamNames={'TT_DATA'; 'TT_COEFF'; 'TT_ACC'; 'NSAMP'}  ClassTemplateParamKinds={'type'; 'type'; 'type'; 'nontype'}  ClassTemplateParamTypes={'typename'; 'typename'; 'typename'; 'unsigned int'}  ClassTemplateParamValues={'cint16', 'cint16', 'cacc48', '2048'}  ClassCtorParamNames={'coeff0_i'; 'coeff1_i'}  ClassCtorParamSerializedTypes={'{R{C{ETT_COEFF}8}}'; '{R{C{ETT_COEFF}8}}'}  ClassCtorParamValues={'[32767 0+32767i -32768 0-32768i -32768 12540-30274i 23170+23170i -30274+12540i]', '[32767 -23170+23170i 0-32768i 23170+23170i -32768 30274-12540i -23170+23170i 12540-30274i]'}  ClassIndex=1  ClassCtorIndex=1  ClassTabVisible=on  ClassTemplateParamsVisible=on  ClassCtorDeclVisible=on  ClassCtorParamsVisible=on  FunctionTabVisible=on  FunctionDecl=|  PortAttrs={ 'input', 'sig0_i', 'input_stream< TT_DATA > * restrict', '', '', '', ''; 'input', 'sig1_i', 'input_stream< TT_DATA > * restrict', '', '', '', ''; 'input', 'acc_i', 'input_stream< TT_ACC > * restrict', '', '', '', ''; 'output', 'acc_o', 'output_stream< TT_ACC > * restrict', '', '', '', '8*N' }  PortAttrsEnables={'off', 'off', 'off', 'off', 'off', 'off', 'off';'off', 'off', 'off', 'off', 'off', 'off', 'off';'off', 'off', 'off', 'off', 'off', 'off', 'off';'off', 'off', 'off', 'off', 'off', 'off', 'on'}  SampleTime=-1  ClassDeclTypeOptions=C[1 1]@t107@template < typename TT_DATA, typename TT_COEFF, typename TT_ACC, unsigned int NSAMP > class dft_1xN_middle;  ClassDecl=template < typename TT_DATA, typename TT_COEFF, typename TT_ACC, unsigned int NSAMP > class dft_1xN_middle;  ClassTemplateParams={ 'TT_DATA', 'typename', 'cint16'; 'TT_COEFF', 'typename', 'cint16'; 'TT_ACC', 'typename', 'cacc48'; 'NSAMP', 'unsigned int', '4*N' }  ClassTemplateParamsEnables={'off', 'off', 'on';'off', 'off', 'on';'off', 'off', 'on';'off', 'off', 'on'}  ClassCtorDeclTypeOptions=C[1 1]@t76@dft_1xN_middle(TT_COEFF ( & coeff0_i ) [ 8 ], TT_COEFF ( & coeff1_i ) [ 8 ])  ClassCtorDecl=dft_1xN_middle(TT_COEFF ( & coeff0_i ) [ 8 ], TT_COEFF ( & coeff1_i ) [ 8 ])  ClassCtorParams={ 'coeff0_i', 'TT_COEFF ( &) [ 8 ]', 'twidC0(2,:)'; 'coeff1_i', 'TT_COEFF ( &) [ 8 ]', 'twidC1(2,:)' }  KernelHeaderFile=aie/dft_1xN_widget.h  KernelClassName=dft_1xN_middle  KernelFunction=run_middle  KernelSourceFile=aie/dft_1xN_widget.cpp  KernelSearchPaths={}  PreProcOptions={}  blockJsonConstraints=[]
      KernelAllAttrs=|
      | s[12;12;9;9;19;14;21;23;21;23;24;21;15;17;12;24;26;26;26;27;28;9;21;23;23;23;24;25;14;19;19;29]@FunctionNameDeclFileNamePortNamesPortTypesPortSerializedTypesPortDirectionsPortWindowSizeEnablesPortWindowMarginEnablesPortBufferSizeEnablesPortBufferMarginEnablesPortSynchronicityEnablesPortSignalSizeEnablesPortBufferSizesPortBufferMarginsFunctionDeclFunctionTemplateSpecKindFunctionTemplateParamNamesFunctionTemplateParamKindsFunctionTemplateParamTypesFunctionTemplateParamValuesFunctionTemplateParamEnablesClassDeclClassTemplateSpecKindClassTemplateParamNamesClassTemplateParamKindsClassTemplateParamTypesClassTemplateParamValuesClassTemplateParamEnablesClassCtorDeclsClassCtorParamNamesClassCtorParamTypesClassCtorParamSerializedTypes[1 1]@C[32 1]@t10@run_middlet22@../../dft_1xN_widget.hC[4 1]@t6@sig0_it6@sig1_it5@acc_it5@acc_oC[4 1]@t34@input_stream< TT_DATA > * restrictt34@input_stream< TT_DATA > * restrictt33@input_stream< TT_ACC > * restrictt34@output_stream< TT_ACC > * restrictC[4 1]@t38@{Q2{P{Tinput_stream{1{t{ETT_DATA}}}}}}t38@{Q2{P{Tinput_stream{1{t{ETT_DATA}}}}}}t37@{Q2{P{Tinput_stream{1{t{ETT_ACC}}}}}}t38@{Q2{P{Toutput_stream{1{t{ETT_ACC}}}}}}C[4 1]@t5@inputt5@inputt5@inputt6@outputC[4 1]@l0@l0@l0@l0@C[4 1]@l0@l0@l0@l0@C[4 1]@l0@l0@l0@l0@C[4 1]@l0@l0@l0@l0@C[4 1]@l0@l0@l0@l0@C[4 1]@l0@l0@l0@l1@C[4 1]@nnnnC[4 1]@nnnnt288@template < typename TT_DATA, typename TT_COEFF, typename TT_ACC, unsigned int NSAMP > 
      | void dft_1xN_middle::
      | run_middle(input_stream< TT_DATA > * restrict sig0_i, input_stream< TT_DATA > * restrict sig1_i, input_stream< TT_ACC > * restrict acc_i, output_stream< TT_ACC > * restrict acc_o)t4@nonee[0 1]@e[0 1]@e[0 1]@e[0 1]@e[0 1]@t107@template < typename TT_DATA, typename TT_COEFF, typename TT_ACC, unsigned int NSAMP > class dft_1xN_middle;t8@implicitC[4 1]@t7@TT_DATAt8@TT_COEFFt6@TT_ACCt5@NSAMPC[4 1]@t4@typet4@typet4@typet7@nontypeC[4 1]@t8@typenamet8@typenamet8@typenamet12@unsigned intC[4 1]@nnnnC[4 1]@l1@l1@l1@l1@C[1 1]@t76@dft_1xN_middle(TT_COEFF ( & coeff0_i ) [ 8 ], TT_COEFF ( & coeff1_i ) [ 8 ])C[1 1]@C[2 1]@t8@coeff0_it8@coeff1_iC[1 1]@C[2 1]@t19@TT_COEFF ( &) [ 8 ]t19@TT_COEFF ( &) [ 8 ]C[1 1]@C[2 1]@t18@{R{C{ETT_COEFF}8}}t18@{R{C{ETT_COEFF}8}}
      FunctionDecl=|
      | template < typename TT_DATA, typename TT_COEFF, typename TT_ACC, unsigned int NSAMP > 
      | void dft_1xN_middle::
      | run_middle(input_stream< TT_DATA > * restrict sig0_i, input_stream< TT_DATA > * restrict sig1_i, input_stream< TT_ACC > * restrict acc_i, output_stream< TT_ACC > * restrict acc_o)
  run_middle5 : aieBasic/AIE Class Kernel  KernelAllAttrs=|  PortNames={'sig0_i'; 'sig1_i'; 'acc_i'; 'acc_o'}  PortSerializedTypes={'{Q2{P{Tinput_stream{1{t{ETT_DATA}}}}}}'; '{Q2{P{Tinput_stream{1{t{ETT_DATA}}}}}}'; '{Q2{P{Tinput_stream{1{t{ETT_ACC}}}}}}'; '{Q2{P{Toutput_stream{1{t{ETT_ACC}}}}}}'}  PortWindowSizes={0.000000000000000000e+00; 0.000000000000000000e+00; 0.000000000000000000e+00; 0.000000000000000000e+00}  PortWindowMargins={0.000000000000000000e+00; 0.000000000000000000e+00; 0.000000000000000000e+00; 0.000000000000000000e+00}  PortSynchronicities={'auto', 'auto', 'auto', 'auto'}  PortSignalSizes={0.000000000000000000e+00; 0.000000000000000000e+00; 0.000000000000000000e+00; 4.096000000000000000e+03}  ClassTemplateSpecKind=implicit  ClassTemplateParamNames={'TT_DATA'; 'TT_COEFF'; 'TT_ACC'; 'NSAMP'}  ClassTemplateParamKinds={'type'; 'type'; 'type'; 'nontype'}  ClassTemplateParamTypes={'typename'; 'typename'; 'typename'; 'unsigned int'}  ClassTemplateParamValues={'cint16', 'cint16', 'cacc48', '2048'}  ClassCtorParamNames={'coeff0_i'; 'coeff1_i'}  ClassCtorParamSerializedTypes={'{R{C{ETT_COEFF}8}}'; '{R{C{ETT_COEFF}8}}'}  ClassCtorParamValues={'[32767 -32768 32767 -32768 -32768 30274+12540i -23170-23170i 12540+30274i]', '[32767 -23170-23170i 0+32767i 23170-23170i -32768 12540+30274i 23170-23170i -30274-12540i]'}  ClassIndex=1  ClassCtorIndex=1  ClassTabVisible=on  ClassTemplateParamsVisible=on  ClassCtorDeclVisible=on  ClassCtorParamsVisible=on  FunctionTabVisible=on  FunctionDecl=|  PortAttrs={ 'input', 'sig0_i', 'input_stream< TT_DATA > * restrict', '', '', '', ''; 'input', 'sig1_i', 'input_stream< TT_DATA > * restrict', '', '', '', ''; 'input', 'acc_i', 'input_stream< TT_ACC > * restrict', '', '', '', ''; 'output', 'acc_o', 'output_stream< TT_ACC > * restrict', '', '', '', '8*N' }  PortAttrsEnables={'off', 'off', 'off', 'off', 'off', 'off', 'off';'off', 'off', 'off', 'off', 'off', 'off', 'off';'off', 'off', 'off', 'off', 'off', 'off', 'off';'off', 'off', 'off', 'off', 'off', 'off', 'on'}  SampleTime=-1  ClassDeclTypeOptions=C[1 1]@t107@template < typename TT_DATA, typename TT_COEFF, typename TT_ACC, unsigned int NSAMP > class dft_1xN_middle;  ClassDecl=template < typename TT_DATA, typename TT_COEFF, typename TT_ACC, unsigned int NSAMP > class dft_1xN_middle;  ClassTemplateParams={ 'TT_DATA', 'typename', 'cint16'; 'TT_COEFF', 'typename', 'cint16'; 'TT_ACC', 'typename', 'cacc48'; 'NSAMP', 'unsigned int', '4*N' }  ClassTemplateParamsEnables={'off', 'off', 'on';'off', 'off', 'on';'off', 'off', 'on';'off', 'off', 'on'}  ClassCtorDeclTypeOptions=C[1 1]@t76@dft_1xN_middle(TT_COEFF ( & coeff0_i ) [ 8 ], TT_COEFF ( & coeff1_i ) [ 8 ])  ClassCtorDecl=dft_1xN_middle(TT_COEFF ( & coeff0_i ) [ 8 ], TT_COEFF ( & coeff1_i ) [ 8 ])  ClassCtorParams={ 'coeff0_i', 'TT_COEFF ( &) [ 8 ]', 'twidC0(3,:)'; 'coeff1_i', 'TT_COEFF ( &) [ 8 ]', 'twidC1(3,:)' }  KernelHeaderFile=aie/dft_1xN_widget.h  KernelClassName=dft_1xN_middle  KernelFunction=run_middle  KernelSourceFile=aie/dft_1xN_widget.cpp  KernelSearchPaths={}  PreProcOptions={}  blockJsonConstraints=[]
      KernelAllAttrs=|
      | s[12;12;9;9;19;14;21;23;21;23;24;21;15;17;12;24;26;26;26;27;28;9;21;23;23;23;24;25;14;19;19;29]@FunctionNameDeclFileNamePortNamesPortTypesPortSerializedTypesPortDirectionsPortWindowSizeEnablesPortWindowMarginEnablesPortBufferSizeEnablesPortBufferMarginEnablesPortSynchronicityEnablesPortSignalSizeEnablesPortBufferSizesPortBufferMarginsFunctionDeclFunctionTemplateSpecKindFunctionTemplateParamNamesFunctionTemplateParamKindsFunctionTemplateParamTypesFunctionTemplateParamValuesFunctionTemplateParamEnablesClassDeclClassTemplateSpecKindClassTemplateParamNamesClassTemplateParamKindsClassTemplateParamTypesClassTemplateParamValuesClassTemplateParamEnablesClassCtorDeclsClassCtorParamNamesClassCtorParamTypesClassCtorParamSerializedTypes[1 1]@C[32 1]@t10@run_middlet22@../../dft_1xN_widget.hC[4 1]@t6@sig0_it6@sig1_it5@acc_it5@acc_oC[4 1]@t34@input_stream< TT_DATA > * restrictt34@input_stream< TT_DATA > * restrictt33@input_stream< TT_ACC > * restrictt34@output_stream< TT_ACC > * restrictC[4 1]@t38@{Q2{P{Tinput_stream{1{t{ETT_DATA}}}}}}t38@{Q2{P{Tinput_stream{1{t{ETT_DATA}}}}}}t37@{Q2{P{Tinput_stream{1{t{ETT_ACC}}}}}}t38@{Q2{P{Toutput_stream{1{t{ETT_ACC}}}}}}C[4 1]@t5@inputt5@inputt5@inputt6@outputC[4 1]@l0@l0@l0@l0@C[4 1]@l0@l0@l0@l0@C[4 1]@l0@l0@l0@l0@C[4 1]@l0@l0@l0@l0@C[4 1]@l0@l0@l0@l0@C[4 1]@l0@l0@l0@l1@C[4 1]@nnnnC[4 1]@nnnnt288@template < typename TT_DATA, typename TT_COEFF, typename TT_ACC, unsigned int NSAMP > 
      | void dft_1xN_middle::
      | run_middle(input_stream< TT_DATA > * restrict sig0_i, input_stream< TT_DATA > * restrict sig1_i, input_stream< TT_ACC > * restrict acc_i, output_stream< TT_ACC > * restrict acc_o)t4@nonee[0 1]@e[0 1]@e[0 1]@e[0 1]@e[0 1]@t107@template < typename TT_DATA, typename TT_COEFF, typename TT_ACC, unsigned int NSAMP > class dft_1xN_middle;t8@implicitC[4 1]@t7@TT_DATAt8@TT_COEFFt6@TT_ACCt5@NSAMPC[4 1]@t4@typet4@typet4@typet7@nontypeC[4 1]@t8@typenamet8@typenamet8@typenamet12@unsigned intC[4 1]@nnnnC[4 1]@l1@l1@l1@l1@C[1 1]@t76@dft_1xN_middle(TT_COEFF ( & coeff0_i ) [ 8 ], TT_COEFF ( & coeff1_i ) [ 8 ])C[1 1]@C[2 1]@t8@coeff0_it8@coeff1_iC[1 1]@C[2 1]@t19@TT_COEFF ( &) [ 8 ]t19@TT_COEFF ( &) [ 8 ]C[1 1]@C[2 1]@t18@{R{C{ETT_COEFF}8}}t18@{R{C{ETT_COEFF}8}}
      FunctionDecl=|
      | template < typename TT_DATA, typename TT_COEFF, typename TT_ACC, unsigned int NSAMP > 
      | void dft_1xN_middle::
      | run_middle(input_stream< TT_DATA > * restrict sig0_i, input_stream< TT_DATA > * restrict sig1_i, input_stream< TT_ACC > * restrict acc_i, output_stream< TT_ACC > * restrict acc_o)
  run_middle6 : aieBasic/AIE Class Kernel  KernelAllAttrs=|  PortNames={'sig0_i'; 'sig1_i'; 'acc_i'; 'acc_o'}  PortSerializedTypes={'{Q2{P{Tinput_stream{1{t{ETT_DATA}}}}}}'; '{Q2{P{Tinput_stream{1{t{ETT_DATA}}}}}}'; '{Q2{P{Tinput_stream{1{t{ETT_ACC}}}}}}'; '{Q2{P{Toutput_stream{1{t{ETT_ACC}}}}}}'}  PortWindowSizes={0.000000000000000000e+00; 0.000000000000000000e+00; 0.000000000000000000e+00; 0.000000000000000000e+00}  PortWindowMargins={0.000000000000000000e+00; 0.000000000000000000e+00; 0.000000000000000000e+00; 0.000000000000000000e+00}  PortSynchronicities={'auto', 'auto', 'auto', 'auto'}  PortSignalSizes={0.000000000000000000e+00; 0.000000000000000000e+00; 0.000000000000000000e+00; 4.096000000000000000e+03}  ClassTemplateSpecKind=implicit  ClassTemplateParamNames={'TT_DATA'; 'TT_COEFF'; 'TT_ACC'; 'NSAMP'}  ClassTemplateParamKinds={'type'; 'type'; 'type'; 'nontype'}  ClassTemplateParamTypes={'typename'; 'typename'; 'typename'; 'unsigned int'}  ClassTemplateParamValues={'cint16', 'cint16', 'cacc48', '2048'}  ClassCtorParamNames={'coeff0_i'; 'coeff1_i'}  ClassCtorParamSerializedTypes={'{R{C{ETT_COEFF}8}}'; '{R{C{ETT_COEFF}8}}'}  ClassCtorParamValues={'[32767 0+32767i -32768 0-32768i 0-32768i 30274+12540i -23170+23170i -12540-30274i]', '[-32768 23170-23170i 0+32767i -23170-23170i 0+32767i -12540-30274i 23170+23170i -30274-12540i]'}  ClassIndex=1  ClassCtorIndex=1  ClassTabVisible=on  ClassTemplateParamsVisible=on  ClassCtorDeclVisible=on  ClassCtorParamsVisible=on  FunctionTabVisible=on  FunctionDecl=|  PortAttrs={ 'input', 'sig0_i', 'input_stream< TT_DATA > * restrict', '', '', '', ''; 'input', 'sig1_i', 'input_stream< TT_DATA > * restrict', '', '', '', ''; 'input', 'acc_i', 'input_stream< TT_ACC > * restrict', '', '', '', ''; 'output', 'acc_o', 'output_stream< TT_ACC > * restrict', '', '', '', '8*N' }  PortAttrsEnables={'off', 'off', 'off', 'off', 'off', 'off', 'off';'off', 'off', 'off', 'off', 'off', 'off', 'off';'off', 'off', 'off', 'off', 'off', 'off', 'off';'off', 'off', 'off', 'off', 'off', 'off', 'on'}  SampleTime=-1  ClassDeclTypeOptions=C[1 1]@t107@template < typename TT_DATA, typename TT_COEFF, typename TT_ACC, unsigned int NSAMP > class dft_1xN_middle;  ClassDecl=template < typename TT_DATA, typename TT_COEFF, typename TT_ACC, unsigned int NSAMP > class dft_1xN_middle;  ClassTemplateParams={ 'TT_DATA', 'typename', 'cint16'; 'TT_COEFF', 'typename', 'cint16'; 'TT_ACC', 'typename', 'cacc48'; 'NSAMP', 'unsigned int', '4*N' }  ClassTemplateParamsEnables={'off', 'off', 'on';'off', 'off', 'on';'off', 'off', 'on';'off', 'off', 'on'}  ClassCtorDeclTypeOptions=C[1 1]@t76@dft_1xN_middle(TT_COEFF ( & coeff0_i ) [ 8 ], TT_COEFF ( & coeff1_i ) [ 8 ])  ClassCtorDecl=dft_1xN_middle(TT_COEFF ( & coeff0_i ) [ 8 ], TT_COEFF ( & coeff1_i ) [ 8 ])  ClassCtorParams={ 'coeff0_i', 'TT_COEFF ( &) [ 8 ]', 'twidD0(2,:)'; 'coeff1_i', 'TT_COEFF ( &) [ 8 ]', 'twidD1(2,:)' }  KernelHeaderFile=aie/dft_1xN_widget.h  KernelClassName=dft_1xN_middle  KernelFunction=run_middle  KernelSourceFile=aie/dft_1xN_widget.cpp  KernelSearchPaths={}  PreProcOptions={}  blockJsonConstraints=[]
      KernelAllAttrs=|
      | s[12;12;9;9;19;14;21;23;21;23;24;21;15;17;12;24;26;26;26;27;28;9;21;23;23;23;24;25;14;19;19;29]@FunctionNameDeclFileNamePortNamesPortTypesPortSerializedTypesPortDirectionsPortWindowSizeEnablesPortWindowMarginEnablesPortBufferSizeEnablesPortBufferMarginEnablesPortSynchronicityEnablesPortSignalSizeEnablesPortBufferSizesPortBufferMarginsFunctionDeclFunctionTemplateSpecKindFunctionTemplateParamNamesFunctionTemplateParamKindsFunctionTemplateParamTypesFunctionTemplateParamValuesFunctionTemplateParamEnablesClassDeclClassTemplateSpecKindClassTemplateParamNamesClassTemplateParamKindsClassTemplateParamTypesClassTemplateParamValuesClassTemplateParamEnablesClassCtorDeclsClassCtorParamNamesClassCtorParamTypesClassCtorParamSerializedTypes[1 1]@C[32 1]@t10@run_middlet22@../../dft_1xN_widget.hC[4 1]@t6@sig0_it6@sig1_it5@acc_it5@acc_oC[4 1]@t34@input_stream< TT_DATA > * restrictt34@input_stream< TT_DATA > * restrictt33@input_stream< TT_ACC > * restrictt34@output_stream< TT_ACC > * restrictC[4 1]@t38@{Q2{P{Tinput_stream{1{t{ETT_DATA}}}}}}t38@{Q2{P{Tinput_stream{1{t{ETT_DATA}}}}}}t37@{Q2{P{Tinput_stream{1{t{ETT_ACC}}}}}}t38@{Q2{P{Toutput_stream{1{t{ETT_ACC}}}}}}C[4 1]@t5@inputt5@inputt5@inputt6@outputC[4 1]@l0@l0@l0@l0@C[4 1]@l0@l0@l0@l0@C[4 1]@l0@l0@l0@l0@C[4 1]@l0@l0@l0@l0@C[4 1]@l0@l0@l0@l0@C[4 1]@l0@l0@l0@l1@C[4 1]@nnnnC[4 1]@nnnnt288@template < typename TT_DATA, typename TT_COEFF, typename TT_ACC, unsigned int NSAMP > 
      | void dft_1xN_middle::
      | run_middle(input_stream< TT_DATA > * restrict sig0_i, input_stream< TT_DATA > * restrict sig1_i, input_stream< TT_ACC > * restrict acc_i, output_stream< TT_ACC > * restrict acc_o)t4@nonee[0 1]@e[0 1]@e[0 1]@e[0 1]@e[0 1]@t107@template < typename TT_DATA, typename TT_COEFF, typename TT_ACC, unsigned int NSAMP > class dft_1xN_middle;t8@implicitC[4 1]@t7@TT_DATAt8@TT_COEFFt6@TT_ACCt5@NSAMPC[4 1]@t4@typet4@typet4@typet7@nontypeC[4 1]@t8@typenamet8@typenamet8@typenamet12@unsigned intC[4 1]@nnnnC[4 1]@l1@l1@l1@l1@C[1 1]@t76@dft_1xN_middle(TT_COEFF ( & coeff0_i ) [ 8 ], TT_COEFF ( & coeff1_i ) [ 8 ])C[1 1]@C[2 1]@t8@coeff0_it8@coeff1_iC[1 1]@C[2 1]@t19@TT_COEFF ( &) [ 8 ]t19@TT_COEFF ( &) [ 8 ]C[1 1]@C[2 1]@t18@{R{C{ETT_COEFF}8}}t18@{R{C{ETT_COEFF}8}}
      FunctionDecl=|
      | template < typename TT_DATA, typename TT_COEFF, typename TT_ACC, unsigned int NSAMP > 
      | void dft_1xN_middle::
      | run_middle(input_stream< TT_DATA > * restrict sig0_i, input_stream< TT_DATA > * restrict sig1_i, input_stream< TT_ACC > * restrict acc_i, output_stream< TT_ACC > * restrict acc_o)
  run_middle7 : aieBasic/AIE Class Kernel  KernelAllAttrs=|  PortNames={'sig0_i'; 'sig1_i'; 'acc_i'; 'acc_o'}  PortSerializedTypes={'{Q2{P{Tinput_stream{1{t{ETT_DATA}}}}}}'; '{Q2{P{Tinput_stream{1{t{ETT_DATA}}}}}}'; '{Q2{P{Tinput_stream{1{t{ETT_ACC}}}}}}'; '{Q2{P{Toutput_stream{1{t{ETT_ACC}}}}}}'}  PortWindowSizes={0.000000000000000000e+00; 0.000000000000000000e+00; 0.000000000000000000e+00; 0.000000000000000000e+00}  PortWindowMargins={0.000000000000000000e+00; 0.000000000000000000e+00; 0.000000000000000000e+00; 0.000000000000000000e+00}  PortSynchronicities={'auto', 'auto', 'auto', 'auto'}  PortSignalSizes={0.000000000000000000e+00; 0.000000000000000000e+00; 0.000000000000000000e+00; 4.096000000000000000e+03}  ClassTemplateSpecKind=implicit  ClassTemplateParamNames={'TT_DATA'; 'TT_COEFF'; 'TT_ACC'; 'NSAMP'}  ClassTemplateParamKinds={'type'; 'type'; 'type'; 'nontype'}  ClassTemplateParamTypes={'typename'; 'typename'; 'typename'; 'unsigned int'}  ClassTemplateParamValues={'cint16', 'cint16', 'cacc48', '2048'}  ClassCtorParamNames={'coeff0_i'; 'coeff1_i'}  ClassCtorParamSerializedTypes={'{R{C{ETT_COEFF}8}}'; '{R{C{ETT_COEFF}8}}'}  ClassCtorParamValues={'[32767 -32768 32767 -32768 0-32768i -12540+30274i 23170-23170i -30274+12540i]', '[-32768 23170+23170i 0-32768i -23170+23170i 0+32767i 30274-12540i -23170-23170i -12540+30274i]'}  ClassIndex=1  ClassCtorIndex=1  ClassTabVisible=on  ClassTemplateParamsVisible=on  ClassCtorDeclVisible=on  ClassCtorParamsVisible=on  FunctionTabVisible=on  FunctionDecl=|  PortAttrs={ 'input', 'sig0_i', 'input_stream< TT_DATA > * restrict', '', '', '', ''; 'input', 'sig1_i', 'input_stream< TT_DATA > * restrict', '', '', '', ''; 'input', 'acc_i', 'input_stream< TT_ACC > * restrict', '', '', '', ''; 'output', 'acc_o', 'output_stream< TT_ACC > * restrict', '', '', '', '8*N' }  PortAttrsEnables={'off', 'off', 'off', 'off', 'off', 'off', 'off';'off', 'off', 'off', 'off', 'off', 'off', 'off';'off', 'off', 'off', 'off', 'off', 'off', 'off';'off', 'off', 'off', 'off', 'off', 'off', 'on'}  SampleTime=-1  ClassDeclTypeOptions=C[1 1]@t107@template < typename TT_DATA, typename TT_COEFF, typename TT_ACC, unsigned int NSAMP > class dft_1xN_middle;  ClassDecl=template < typename TT_DATA, typename TT_COEFF, typename TT_ACC, unsigned int NSAMP > class dft_1xN_middle;  ClassTemplateParams={ 'TT_DATA', 'typename', 'cint16'; 'TT_COEFF', 'typename', 'cint16'; 'TT_ACC', 'typename', 'cacc48'; 'NSAMP', 'unsigned int', '4*N' }  ClassTemplateParamsEnables={'off', 'off', 'on';'off', 'off', 'on';'off', 'off', 'on';'off', 'off', 'on'}  ClassCtorDeclTypeOptions=C[1 1]@t76@dft_1xN_middle(TT_COEFF ( & coeff0_i ) [ 8 ], TT_COEFF ( & coeff1_i ) [ 8 ])  ClassCtorDecl=dft_1xN_middle(TT_COEFF ( & coeff0_i ) [ 8 ], TT_COEFF ( & coeff1_i ) [ 8 ])  ClassCtorParams={ 'coeff0_i', 'TT_COEFF ( &) [ 8 ]', 'twidD0(3,:)'; 'coeff1_i', 'TT_COEFF ( &) [ 8 ]', 'twidD1(3,:)' }  KernelHeaderFile=aie/dft_1xN_widget.h  KernelClassName=dft_1xN_middle  KernelFunction=run_middle  KernelSourceFile=aie/dft_1xN_widget.cpp  KernelSearchPaths={}  PreProcOptions={}  blockJsonConstraints=[]
      KernelAllAttrs=|
      | s[12;12;9;9;19;14;21;23;21;23;24;21;15;17;12;24;26;26;26;27;28;9;21;23;23;23;24;25;14;19;19;29]@FunctionNameDeclFileNamePortNamesPortTypesPortSerializedTypesPortDirectionsPortWindowSizeEnablesPortWindowMarginEnablesPortBufferSizeEnablesPortBufferMarginEnablesPortSynchronicityEnablesPortSignalSizeEnablesPortBufferSizesPortBufferMarginsFunctionDeclFunctionTemplateSpecKindFunctionTemplateParamNamesFunctionTemplateParamKindsFunctionTemplateParamTypesFunctionTemplateParamValuesFunctionTemplateParamEnablesClassDeclClassTemplateSpecKindClassTemplateParamNamesClassTemplateParamKindsClassTemplateParamTypesClassTemplateParamValuesClassTemplateParamEnablesClassCtorDeclsClassCtorParamNamesClassCtorParamTypesClassCtorParamSerializedTypes[1 1]@C[32 1]@t10@run_middlet22@../../dft_1xN_widget.hC[4 1]@t6@sig0_it6@sig1_it5@acc_it5@acc_oC[4 1]@t34@input_stream< TT_DATA > * restrictt34@input_stream< TT_DATA > * restrictt33@input_stream< TT_ACC > * restrictt34@output_stream< TT_ACC > * restrictC[4 1]@t38@{Q2{P{Tinput_stream{1{t{ETT_DATA}}}}}}t38@{Q2{P{Tinput_stream{1{t{ETT_DATA}}}}}}t37@{Q2{P{Tinput_stream{1{t{ETT_ACC}}}}}}t38@{Q2{P{Toutput_stream{1{t{ETT_ACC}}}}}}C[4 1]@t5@inputt5@inputt5@inputt6@outputC[4 1]@l0@l0@l0@l0@C[4 1]@l0@l0@l0@l0@C[4 1]@l0@l0@l0@l0@C[4 1]@l0@l0@l0@l0@C[4 1]@l0@l0@l0@l0@C[4 1]@l0@l0@l0@l1@C[4 1]@nnnnC[4 1]@nnnnt288@template < typename TT_DATA, typename TT_COEFF, typename TT_ACC, unsigned int NSAMP > 
      | void dft_1xN_middle::
      | run_middle(input_stream< TT_DATA > * restrict sig0_i, input_stream< TT_DATA > * restrict sig1_i, input_stream< TT_ACC > * restrict acc_i, output_stream< TT_ACC > * restrict acc_o)t4@nonee[0 1]@e[0 1]@e[0 1]@e[0 1]@e[0 1]@t107@template < typename TT_DATA, typename TT_COEFF, typename TT_ACC, unsigned int NSAMP > class dft_1xN_middle;t8@implicitC[4 1]@t7@TT_DATAt8@TT_COEFFt6@TT_ACCt5@NSAMPC[4 1]@t4@typet4@typet4@typet7@nontypeC[4 1]@t8@typenamet8@typenamet8@typenamet12@unsigned intC[4 1]@nnnnC[4 1]@l1@l1@l1@l1@C[1 1]@t76@dft_1xN_middle(TT_COEFF ( & coeff0_i ) [ 8 ], TT_COEFF ( & coeff1_i ) [ 8 ])C[1 1]@C[2 1]@t8@coeff0_it8@coeff1_iC[1 1]@C[2 1]@t19@TT_COEFF ( &) [ 8 ]t19@TT_COEFF ( &) [ 8 ]C[1 1]@C[2 1]@t18@{R{C{ETT_COEFF}8}}t18@{R{C{ETT_COEFF}8}}
      FunctionDecl=|
      | template < typename TT_DATA, typename TT_COEFF, typename TT_ACC, unsigned int NSAMP > 
      | void dft_1xN_middle::
      | run_middle(input_stream< TT_DATA > * restrict sig0_i, input_stream< TT_DATA > * restrict sig1_i, input_stream< TT_ACC > * restrict acc_i, output_stream< TT_ACC > * restrict acc_o)
  run_output : aieBasic/AIE Class Kernel  KernelAllAttrs=|  PortNames={'sig0_i'; 'sig1_i'; 'acc_i'; 'sig0_o'; 'sig1_o'}  PortSerializedTypes={'{Q2{P{Tinput_stream{1{t{ETT_DATA}}}}}}'; '{Q2{P{Tinput_stream{1{t{ETT_DATA}}}}}}'; '{Q2{P{Tinput_stream{1{t{ETT_ACC}}}}}}'; '{Q2{P{Toutput_stream{1{t{ETT_DATA}}}}}}'; '{Q2{P{Toutput_stream{1{t{ETT_DATA}}}}}}'}  PortWindowSizes={0.000000000000000000e+00; 0.000000000000000000e+00; 0.000000000000000000e+00; 0.000000000000000000e+00; 0.000000000000000000e+00}  PortWindowMargins={0.000000000000000000e+00; 0.000000000000000000e+00; 0.000000000000000000e+00; 0.000000000000000000e+00; 0.000000000000000000e+00}  PortSynchronicities={'auto', 'auto', 'auto', 'auto', 'auto'}  PortSignalSizes={0.000000000000000000e+00; 0.000000000000000000e+00; 0.000000000000000000e+00; 2.048000000000000000e+03; 2.048000000000000000e+03}  ClassTemplateSpecKind=implicit  ClassTemplateParamNames={'TT_DATA'; 'TT_COEFF'; 'TT_ACC'; 'NSAMP'}  ClassTemplateParamKinds={'type'; 'type'; 'type'; 'nontype'}  ClassTemplateParamTypes={'typename'; 'typename'; 'typename'; 'unsigned int'}  ClassTemplateParamValues={'cint16', 'cint16', 'cacc48', '2048'}  ClassCtorParamNames={'coeff0_i'; 'coeff1_i'}  ClassCtorParamSerializedTypes={'{R{C{ETT_COEFF}8}}'; '{R{C{ETT_COEFF}8}}'}  ClassCtorParamValues={'[32767 0-32768i -32768 0+32767i 32767 12540-30274i -23170-23170i -30274+12540i]', '[32767 23170-23170i 0-32768i -23170-23170i 32767 30274-12540i 23170-23170i 12540-30274i]'}  ClassIndex=1  ClassCtorIndex=1  ClassTabVisible=on  ClassTemplateParamsVisible=on  ClassCtorDeclVisible=on  ClassCtorParamsVisible=on  FunctionTabVisible=on  FunctionDecl=|  PortAttrs={ 'input', 'sig0_i', 'input_stream< TT_DATA > * restrict', '', '', '', ''; 'input', 'sig1_i', 'input_stream< TT_DATA > * restrict', '', '', '', ''; 'input', 'acc_i', 'input_stream< TT_ACC > * restrict', '', '', '', ''; 'output', 'sig0_o', 'output_stream< TT_DATA > * restrict', '', '', '', '4*N'; 'output', 'sig1_o', 'output_stream< TT_DATA > * restrict', '', '', '', '4*N' }  PortAttrsEnables={'off', 'off', 'off', 'off', 'off', 'off', 'off';'off', 'off', 'off', 'off', 'off', 'off', 'off';'off', 'off', 'off', 'off', 'off', 'off', 'off';'off', 'off', 'off', 'off', 'off', 'off', 'on';'off', 'off', 'off', 'off', 'off', 'off', 'on'}  SampleTime=-1  ClassDeclTypeOptions=C[1 1]@t107@template < typename TT_DATA, typename TT_COEFF, typename TT_ACC, unsigned int NSAMP > class dft_1xN_output;  ClassDecl=template < typename TT_DATA, typename TT_COEFF, typename TT_ACC, unsigned int NSAMP > class dft_1xN_output;  ClassTemplateParams={ 'TT_DATA', 'typename', 'cint16'; 'TT_COEFF', 'typename', 'cint16'; 'TT_ACC', 'typename', 'cacc48'; 'NSAMP', 'unsigned int', '4*N' }  ClassTemplateParamsEnables={'off', 'off', 'on';'off', 'off', 'on';'off', 'off', 'on';'off', 'off', 'on'}  ClassCtorDeclTypeOptions=C[1 1]@t76@dft_1xN_output(TT_COEFF ( & coeff0_i ) [ 8 ], TT_COEFF ( & coeff1_i ) [ 8 ])  ClassCtorDecl=dft_1xN_output(TT_COEFF ( & coeff0_i ) [ 8 ], TT_COEFF ( & coeff1_i ) [ 8 ])  ClassCtorParams={ 'coeff0_i', 'TT_COEFF ( &) [ 8 ]', 'twidA0(4,:)'; 'coeff1_i', 'TT_COEFF ( &) [ 8 ]', 'twidA1(4,:)' }  KernelHeaderFile=aie/dft_1xN_widget.h  KernelClassName=dft_1xN_output  KernelFunction=run_output  KernelSourceFile=aie/dft_1xN_widget.cpp  KernelSearchPaths={}  PreProcOptions={}  blockJsonConstraints=[]
      KernelAllAttrs=|
      | s[12;12;9;9;19;14;21;23;21;23;24;21;15;17;12;24;26;26;26;27;28;9;21;23;23;23;24;25;14;19;19;29]@FunctionNameDeclFileNamePortNamesPortTypesPortSerializedTypesPortDirectionsPortWindowSizeEnablesPortWindowMarginEnablesPortBufferSizeEnablesPortBufferMarginEnablesPortSynchronicityEnablesPortSignalSizeEnablesPortBufferSizesPortBufferMarginsFunctionDeclFunctionTemplateSpecKindFunctionTemplateParamNamesFunctionTemplateParamKindsFunctionTemplateParamTypesFunctionTemplateParamValuesFunctionTemplateParamEnablesClassDeclClassTemplateSpecKindClassTemplateParamNamesClassTemplateParamKindsClassTemplateParamTypesClassTemplateParamValuesClassTemplateParamEnablesClassCtorDeclsClassCtorParamNamesClassCtorParamTypesClassCtorParamSerializedTypes[1 1]@C[32 1]@t10@run_outputt22@../../dft_1xN_widget.hC[5 1]@t6@sig0_it6@sig1_it5@acc_it6@sig0_ot6@sig1_oC[5 1]@t34@input_stream< TT_DATA > * restrictt34@input_stream< TT_DATA > * restrictt33@input_stream< TT_ACC > * restrictt35@output_stream< TT_DATA > * restrictt35@output_stream< TT_DATA > * restrictC[5 1]@t38@{Q2{P{Tinput_stream{1{t{ETT_DATA}}}}}}t38@{Q2{P{Tinput_stream{1{t{ETT_DATA}}}}}}t37@{Q2{P{Tinput_stream{1{t{ETT_ACC}}}}}}t39@{Q2{P{Toutput_stream{1{t{ETT_DATA}}}}}}t39@{Q2{P{Toutput_stream{1{t{ETT_DATA}}}}}}C[5 1]@t5@inputt5@inputt5@inputt6@outputt6@outputC[5 1]@l0@l0@l0@l0@l0@C[5 1]@l0@l0@l0@l0@l0@C[5 1]@l0@l0@l0@l0@l0@C[5 1]@l0@l0@l0@l0@l0@C[5 1]@l0@l0@l0@l0@l0@C[5 1]@l0@l0@l0@l1@l1@C[5 1]@nnnnnC[5 1]@nnnnnt334@template < typename TT_DATA, typename TT_COEFF, typename TT_ACC, unsigned int NSAMP > 
      | void dft_1xN_output::
      | run_output(input_stream< TT_DATA > * restrict sig0_i, input_stream< TT_DATA > * restrict sig1_i, input_stream< TT_ACC > * restrict acc_i, output_stream< TT_DATA > * restrict sig0_o, output_stream< TT_DATA > * restrict sig1_o)t4@nonee[0 1]@e[0 1]@e[0 1]@e[0 1]@e[0 1]@t107@template < typename TT_DATA, typename TT_COEFF, typename TT_ACC, unsigned int NSAMP > class dft_1xN_output;t8@implicitC[4 1]@t7@TT_DATAt8@TT_COEFFt6@TT_ACCt5@NSAMPC[4 1]@t4@typet4@typet4@typet7@nontypeC[4 1]@t8@typenamet8@typenamet8@typenamet12@unsigned intC[4 1]@nnnnC[4 1]@l1@l1@l1@l1@C[1 1]@t76@dft_1xN_output(TT_COEFF ( & coeff0_i ) [ 8 ], TT_COEFF ( & coeff1_i ) [ 8 ])C[1 1]@C[2 1]@t8@coeff0_it8@coeff1_iC[1 1]@C[2 1]@t19@TT_COEFF ( &) [ 8 ]t19@TT_COEFF ( &) [ 8 ]C[1 1]@C[2 1]@t18@{R{C{ETT_COEFF}8}}t18@{R{C{ETT_COEFF}8}}
      FunctionDecl=|
      | template < typename TT_DATA, typename TT_COEFF, typename TT_ACC, unsigned int NSAMP > 
      | void dft_1xN_output::
      | run_output(input_stream< TT_DATA > * restrict sig0_i, input_stream< TT_DATA > * restrict sig1_i, input_stream< TT_ACC > * restrict acc_i, output_stream< TT_DATA > * restrict sig0_o, output_stream< TT_DATA > * restrict sig1_o)
  run_output1 : aieBasic/AIE Class Kernel  KernelAllAttrs=|  PortNames={'sig0_i'; 'sig1_i'; 'acc_i'; 'sig0_o'; 'sig1_o'}  PortSerializedTypes={'{Q2{P{Tinput_stream{1{t{ETT_DATA}}}}}}'; '{Q2{P{Tinput_stream{1{t{ETT_DATA}}}}}}'; '{Q2{P{Tinput_stream{1{t{ETT_ACC}}}}}}'; '{Q2{P{Toutput_stream{1{t{ETT_DATA}}}}}}'; '{Q2{P{Toutput_stream{1{t{ETT_DATA}}}}}}'}  PortWindowSizes={0.000000000000000000e+00; 0.000000000000000000e+00; 0.000000000000000000e+00; 0.000000000000000000e+00; 0.000000000000000000e+00}  PortWindowMargins={0.000000000000000000e+00; 0.000000000000000000e+00; 0.000000000000000000e+00; 0.000000000000000000e+00; 0.000000000000000000e+00}  PortSynchronicities={'auto', 'auto', 'auto', 'auto', 'auto'}  PortSignalSizes={0.000000000000000000e+00; 0.000000000000000000e+00; 0.000000000000000000e+00; 2.048000000000000000e+03; 2.048000000000000000e+03}  ClassTemplateSpecKind=implicit  ClassTemplateParamNames={'TT_DATA'; 'TT_COEFF'; 'TT_ACC'; 'NSAMP'}  ClassTemplateParamKinds={'type'; 'type'; 'type'; 'nontype'}  ClassTemplateParamTypes={'typename'; 'typename'; 'typename'; 'unsigned int'}  ClassTemplateParamValues={'cint16', 'cint16', 'cacc48', '2048'}  ClassCtorParamNames={'coeff0_i'; 'coeff1_i'}  ClassCtorParamSerializedTypes={'{R{C{ETT_COEFF}8}}'; '{R{C{ETT_COEFF}8}}'}  ClassCtorParamValues={'[32767 0-32768i -32768 0+32767i 0+32767i 30274+12540i 23170-23170i -12540-30274i]', '[-32768 -23170+23170i 0+32767i 23170+23170i 0-32768i -12540-30274i -23170-23170i -30274-12540i]'}  ClassIndex=1  ClassCtorIndex=1  ClassTabVisible=on  ClassTemplateParamsVisible=on  ClassCtorDeclVisible=on  ClassCtorParamsVisible=on  FunctionTabVisible=on  FunctionDecl=|  PortAttrs={ 'input', 'sig0_i', 'input_stream< TT_DATA > * restrict', '', '', '', ''; 'input', 'sig1_i', 'input_stream< TT_DATA > * restrict', '', '', '', ''; 'input', 'acc_i', 'input_stream< TT_ACC > * restrict', '', '', '', ''; 'output', 'sig0_o', 'output_stream< TT_DATA > * restrict', '', '', '', '4*N'; 'output', 'sig1_o', 'output_stream< TT_DATA > * restrict', '', '', '', '4*N' }  PortAttrsEnables={'off', 'off', 'off', 'off', 'off', 'off', 'off';'off', 'off', 'off', 'off', 'off', 'off', 'off';'off', 'off', 'off', 'off', 'off', 'off', 'off';'off', 'off', 'off', 'off', 'off', 'off', 'on';'off', 'off', 'off', 'off', 'off', 'off', 'on'}  SampleTime=-1  ClassDeclTypeOptions=C[1 1]@t107@template < typename TT_DATA, typename TT_COEFF, typename TT_ACC, unsigned int NSAMP > class dft_1xN_output;  ClassDecl=template < typename TT_DATA, typename TT_COEFF, typename TT_ACC, unsigned int NSAMP > class dft_1xN_output;  ClassTemplateParams={ 'TT_DATA', 'typename', 'cint16'; 'TT_COEFF', 'typename', 'cint16'; 'TT_ACC', 'typename', 'cacc48'; 'NSAMP', 'unsigned int', '4*N' }  ClassTemplateParamsEnables={'off', 'off', 'on';'off', 'off', 'on';'off', 'off', 'on';'off', 'off', 'on'}  ClassCtorDeclTypeOptions=C[1 1]@t76@dft_1xN_output(TT_COEFF ( & coeff0_i ) [ 8 ], TT_COEFF ( & coeff1_i ) [ 8 ])  ClassCtorDecl=dft_1xN_output(TT_COEFF ( & coeff0_i ) [ 8 ], TT_COEFF ( & coeff1_i ) [ 8 ])  ClassCtorParams={ 'coeff0_i', 'TT_COEFF ( &) [ 8 ]', 'twidB0(4,:)'; 'coeff1_i', 'TT_COEFF ( &) [ 8 ]', 'twidB1(4,:)' }  KernelHeaderFile=aie/dft_1xN_widget.h  KernelClassName=dft_1xN_output  KernelFunction=run_output  KernelSourceFile=aie/dft_1xN_widget.cpp  KernelSearchPaths={}  PreProcOptions={}  blockJsonConstraints=[]
      KernelAllAttrs=|
      | s[12;12;9;9;19;14;21;23;21;23;24;21;15;17;12;24;26;26;26;27;28;9;21;23;23;23;24;25;14;19;19;29]@FunctionNameDeclFileNamePortNamesPortTypesPortSerializedTypesPortDirectionsPortWindowSizeEnablesPortWindowMarginEnablesPortBufferSizeEnablesPortBufferMarginEnablesPortSynchronicityEnablesPortSignalSizeEnablesPortBufferSizesPortBufferMarginsFunctionDeclFunctionTemplateSpecKindFunctionTemplateParamNamesFunctionTemplateParamKindsFunctionTemplateParamTypesFunctionTemplateParamValuesFunctionTemplateParamEnablesClassDeclClassTemplateSpecKindClassTemplateParamNamesClassTemplateParamKindsClassTemplateParamTypesClassTemplateParamValuesClassTemplateParamEnablesClassCtorDeclsClassCtorParamNamesClassCtorParamTypesClassCtorParamSerializedTypes[1 1]@C[32 1]@t10@run_outputt22@../../dft_1xN_widget.hC[5 1]@t6@sig0_it6@sig1_it5@acc_it6@sig0_ot6@sig1_oC[5 1]@t34@input_stream< TT_DATA > * restrictt34@input_stream< TT_DATA > * restrictt33@input_stream< TT_ACC > * restrictt35@output_stream< TT_DATA > * restrictt35@output_stream< TT_DATA > * restrictC[5 1]@t38@{Q2{P{Tinput_stream{1{t{ETT_DATA}}}}}}t38@{Q2{P{Tinput_stream{1{t{ETT_DATA}}}}}}t37@{Q2{P{Tinput_stream{1{t{ETT_ACC}}}}}}t39@{Q2{P{Toutput_stream{1{t{ETT_DATA}}}}}}t39@{Q2{P{Toutput_stream{1{t{ETT_DATA}}}}}}C[5 1]@t5@inputt5@inputt5@inputt6@outputt6@outputC[5 1]@l0@l0@l0@l0@l0@C[5 1]@l0@l0@l0@l0@l0@C[5 1]@l0@l0@l0@l0@l0@C[5 1]@l0@l0@l0@l0@l0@C[5 1]@l0@l0@l0@l0@l0@C[5 1]@l0@l0@l0@l1@l1@C[5 1]@nnnnnC[5 1]@nnnnnt334@template < typename TT_DATA, typename TT_COEFF, typename TT_ACC, unsigned int NSAMP > 
      | void dft_1xN_output::
      | run_output(input_stream< TT_DATA > * restrict sig0_i, input_stream< TT_DATA > * restrict sig1_i, input_stream< TT_ACC > * restrict acc_i, output_stream< TT_DATA > * restrict sig0_o, output_stream< TT_DATA > * restrict sig1_o)t4@nonee[0 1]@e[0 1]@e[0 1]@e[0 1]@e[0 1]@t107@template < typename TT_DATA, typename TT_COEFF, typename TT_ACC, unsigned int NSAMP > class dft_1xN_output;t8@implicitC[4 1]@t7@TT_DATAt8@TT_COEFFt6@TT_ACCt5@NSAMPC[4 1]@t4@typet4@typet4@typet7@nontypeC[4 1]@t8@typenamet8@typenamet8@typenamet12@unsigned intC[4 1]@nnnnC[4 1]@l1@l1@l1@l1@C[1 1]@t76@dft_1xN_output(TT_COEFF ( & coeff0_i ) [ 8 ], TT_COEFF ( & coeff1_i ) [ 8 ])C[1 1]@C[2 1]@t8@coeff0_it8@coeff1_iC[1 1]@C[2 1]@t19@TT_COEFF ( &) [ 8 ]t19@TT_COEFF ( &) [ 8 ]C[1 1]@C[2 1]@t18@{R{C{ETT_COEFF}8}}t18@{R{C{ETT_COEFF}8}}
      FunctionDecl=|
      | template < typename TT_DATA, typename TT_COEFF, typename TT_ACC, unsigned int NSAMP > 
      | void dft_1xN_output::
      | run_output(input_stream< TT_DATA > * restrict sig0_i, input_stream< TT_DATA > * restrict sig1_i, input_stream< TT_ACC > * restrict acc_i, output_stream< TT_DATA > * restrict sig0_o, output_stream< TT_DATA > * restrict sig1_o)
  run_output2 : aieBasic/AIE Class Kernel  KernelAllAttrs=|  PortNames={'sig0_i'; 'sig1_i'; 'acc_i'; 'sig0_o'; 'sig1_o'}  PortSerializedTypes={'{Q2{P{Tinput_stream{1{t{ETT_DATA}}}}}}'; '{Q2{P{Tinput_stream{1{t{ETT_DATA}}}}}}'; '{Q2{P{Tinput_stream{1{t{ETT_ACC}}}}}}'; '{Q2{P{Toutput_stream{1{t{ETT_DATA}}}}}}'; '{Q2{P{Toutput_stream{1{t{ETT_DATA}}}}}}'}  PortWindowSizes={0.000000000000000000e+00; 0.000000000000000000e+00; 0.000000000000000000e+00; 0.000000000000000000e+00; 0.000000000000000000e+00}  PortWindowMargins={0.000000000000000000e+00; 0.000000000000000000e+00; 0.000000000000000000e+00; 0.000000000000000000e+00; 0.000000000000000000e+00}  PortSynchronicities={'auto', 'auto', 'auto', 'auto', 'auto'}  PortSignalSizes={0.000000000000000000e+00; 0.000000000000000000e+00; 0.000000000000000000e+00; 2.048000000000000000e+03; 2.048000000000000000e+03}  ClassTemplateSpecKind=implicit  ClassTemplateParamNames={'TT_DATA'; 'TT_COEFF'; 'TT_ACC'; 'NSAMP'}  ClassTemplateParamKinds={'type'; 'type'; 'type'; 'nontype'}  ClassTemplateParamTypes={'typename'; 'typename'; 'typename'; 'unsigned int'}  ClassTemplateParamValues={'cint16', 'cint16', 'cacc48', '2048'}  ClassCtorParamNames={'coeff0_i'; 'coeff1_i'}  ClassCtorParamSerializedTypes={'{R{C{ETT_COEFF}8}}'; '{R{C{ETT_COEFF}8}}'}  ClassCtorParamValues={'[32767 0-32768i -32768 0+32767i -32768 -12540+30274i 23170+23170i 30274-12540i]', '[32767 23170-23170i 0-32768i -23170-23170i -32768 -30274+12540i -23170+23170i -12540+30274i]'}  ClassIndex=1  ClassCtorIndex=1  ClassTabVisible=on  ClassTemplateParamsVisible=on  ClassCtorDeclVisible=on  ClassCtorParamsVisible=on  FunctionTabVisible=on  FunctionDecl=|  PortAttrs={ 'input', 'sig0_i', 'input_stream< TT_DATA > * restrict', '', '', '', ''; 'input', 'sig1_i', 'input_stream< TT_DATA > * restrict', '', '', '', ''; 'input', 'acc_i', 'input_stream< TT_ACC > * restrict', '', '', '', ''; 'output', 'sig0_o', 'output_stream< TT_DATA > * restrict', '', '', '', '4*N'; 'output', 'sig1_o', 'output_stream< TT_DATA > * restrict', '', '', '', '4*N' }  PortAttrsEnables={'off', 'off', 'off', 'off', 'off', 'off', 'off';'off', 'off', 'off', 'off', 'off', 'off', 'off';'off', 'off', 'off', 'off', 'off', 'off', 'off';'off', 'off', 'off', 'off', 'off', 'off', 'on';'off', 'off', 'off', 'off', 'off', 'off', 'on'}  SampleTime=-1  ClassDeclTypeOptions=C[1 1]@t107@template < typename TT_DATA, typename TT_COEFF, typename TT_ACC, unsigned int NSAMP > class dft_1xN_output;  ClassDecl=template < typename TT_DATA, typename TT_COEFF, typename TT_ACC, unsigned int NSAMP > class dft_1xN_output;  ClassTemplateParams={ 'TT_DATA', 'typename', 'cint16'; 'TT_COEFF', 'typename', 'cint16'; 'TT_ACC', 'typename', 'cacc48'; 'NSAMP', 'unsigned int', '4*N' }  ClassTemplateParamsEnables={'off', 'off', 'on';'off', 'off', 'on';'off', 'off', 'on';'off', 'off', 'on'}  ClassCtorDeclTypeOptions=C[1 1]@t76@dft_1xN_output(TT_COEFF ( & coeff0_i ) [ 8 ], TT_COEFF ( & coeff1_i ) [ 8 ])  ClassCtorDecl=dft_1xN_output(TT_COEFF ( & coeff0_i ) [ 8 ], TT_COEFF ( & coeff1_i ) [ 8 ])  ClassCtorParams={ 'coeff0_i', 'TT_COEFF ( &) [ 8 ]', 'twidC0(4,:)'; 'coeff1_i', 'TT_COEFF ( &) [ 8 ]', 'twidC1(4,:)' }  KernelHeaderFile=aie/dft_1xN_widget.h  KernelClassName=dft_1xN_output  KernelFunction=run_output  KernelSourceFile=aie/dft_1xN_widget.cpp  KernelSearchPaths={}  PreProcOptions={}  blockJsonConstraints=[]
      KernelAllAttrs=|
      | s[12;12;9;9;19;14;21;23;21;23;24;21;15;17;12;24;26;26;26;27;28;9;21;23;23;23;24;25;14;19;19;29]@FunctionNameDeclFileNamePortNamesPortTypesPortSerializedTypesPortDirectionsPortWindowSizeEnablesPortWindowMarginEnablesPortBufferSizeEnablesPortBufferMarginEnablesPortSynchronicityEnablesPortSignalSizeEnablesPortBufferSizesPortBufferMarginsFunctionDeclFunctionTemplateSpecKindFunctionTemplateParamNamesFunctionTemplateParamKindsFunctionTemplateParamTypesFunctionTemplateParamValuesFunctionTemplateParamEnablesClassDeclClassTemplateSpecKindClassTemplateParamNamesClassTemplateParamKindsClassTemplateParamTypesClassTemplateParamValuesClassTemplateParamEnablesClassCtorDeclsClassCtorParamNamesClassCtorParamTypesClassCtorParamSerializedTypes[1 1]@C[32 1]@t10@run_outputt22@../../dft_1xN_widget.hC[5 1]@t6@sig0_it6@sig1_it5@acc_it6@sig0_ot6@sig1_oC[5 1]@t34@input_stream< TT_DATA > * restrictt34@input_stream< TT_DATA > * restrictt33@input_stream< TT_ACC > * restrictt35@output_stream< TT_DATA > * restrictt35@output_stream< TT_DATA > * restrictC[5 1]@t38@{Q2{P{Tinput_stream{1{t{ETT_DATA}}}}}}t38@{Q2{P{Tinput_stream{1{t{ETT_DATA}}}}}}t37@{Q2{P{Tinput_stream{1{t{ETT_ACC}}}}}}t39@{Q2{P{Toutput_stream{1{t{ETT_DATA}}}}}}t39@{Q2{P{Toutput_stream{1{t{ETT_DATA}}}}}}C[5 1]@t5@inputt5@inputt5@inputt6@outputt6@outputC[5 1]@l0@l0@l0@l0@l0@C[5 1]@l0@l0@l0@l0@l0@C[5 1]@l0@l0@l0@l0@l0@C[5 1]@l0@l0@l0@l0@l0@C[5 1]@l0@l0@l0@l0@l0@C[5 1]@l0@l0@l0@l1@l1@C[5 1]@nnnnnC[5 1]@nnnnnt334@template < typename TT_DATA, typename TT_COEFF, typename TT_ACC, unsigned int NSAMP > 
      | void dft_1xN_output::
      | run_output(input_stream< TT_DATA > * restrict sig0_i, input_stream< TT_DATA > * restrict sig1_i, input_stream< TT_ACC > * restrict acc_i, output_stream< TT_DATA > * restrict sig0_o, output_stream< TT_DATA > * restrict sig1_o)t4@nonee[0 1]@e[0 1]@e[0 1]@e[0 1]@e[0 1]@t107@template < typename TT_DATA, typename TT_COEFF, typename TT_ACC, unsigned int NSAMP > class dft_1xN_output;t8@implicitC[4 1]@t7@TT_DATAt8@TT_COEFFt6@TT_ACCt5@NSAMPC[4 1]@t4@typet4@typet4@typet7@nontypeC[4 1]@t8@typenamet8@typenamet8@typenamet12@unsigned intC[4 1]@nnnnC[4 1]@l1@l1@l1@l1@C[1 1]@t76@dft_1xN_output(TT_COEFF ( & coeff0_i ) [ 8 ], TT_COEFF ( & coeff1_i ) [ 8 ])C[1 1]@C[2 1]@t8@coeff0_it8@coeff1_iC[1 1]@C[2 1]@t19@TT_COEFF ( &) [ 8 ]t19@TT_COEFF ( &) [ 8 ]C[1 1]@C[2 1]@t18@{R{C{ETT_COEFF}8}}t18@{R{C{ETT_COEFF}8}}
      FunctionDecl=|
      | template < typename TT_DATA, typename TT_COEFF, typename TT_ACC, unsigned int NSAMP > 
      | void dft_1xN_output::
      | run_output(input_stream< TT_DATA > * restrict sig0_i, input_stream< TT_DATA > * restrict sig1_i, input_stream< TT_ACC > * restrict acc_i, output_stream< TT_DATA > * restrict sig0_o, output_stream< TT_DATA > * restrict sig1_o)
  run_output3 : aieBasic/AIE Class Kernel  KernelAllAttrs=|  PortNames={'sig0_i'; 'sig1_i'; 'acc_i'; 'sig0_o'; 'sig1_o'}  PortSerializedTypes={'{Q2{P{Tinput_stream{1{t{ETT_DATA}}}}}}'; '{Q2{P{Tinput_stream{1{t{ETT_DATA}}}}}}'; '{Q2{P{Tinput_stream{1{t{ETT_ACC}}}}}}'; '{Q2{P{Toutput_stream{1{t{ETT_DATA}}}}}}'; '{Q2{P{Toutput_stream{1{t{ETT_DATA}}}}}}'}  PortWindowSizes={0.000000000000000000e+00; 0.000000000000000000e+00; 0.000000000000000000e+00; 0.000000000000000000e+00; 0.000000000000000000e+00}  PortWindowMargins={0.000000000000000000e+00; 0.000000000000000000e+00; 0.000000000000000000e+00; 0.000000000000000000e+00; 0.000000000000000000e+00}  PortSynchronicities={'auto', 'auto', 'auto', 'auto', 'auto'}  PortSignalSizes={0.000000000000000000e+00; 0.000000000000000000e+00; 0.000000000000000000e+00; 2.048000000000000000e+03; 2.048000000000000000e+03}  ClassTemplateSpecKind=implicit  ClassTemplateParamNames={'TT_DATA'; 'TT_COEFF'; 'TT_ACC'; 'NSAMP'}  ClassTemplateParamKinds={'type'; 'type'; 'type'; 'nontype'}  ClassTemplateParamTypes={'typename'; 'typename'; 'typename'; 'unsigned int'}  ClassTemplateParamValues={'cint16', 'cint16', 'cacc48', '2048'}  ClassCtorParamNames={'coeff0_i'; 'coeff1_i'}  ClassCtorParamSerializedTypes={'{R{C{ETT_COEFF}8}}'; '{R{C{ETT_COEFF}8}}'}  ClassCtorParamValues={'[32767 0-32768i -32768 0+32767i 0-32768i -30274-12540i -23170+23170i 12540+30274i]', '[-32768 -23170+23170i 0+32767i 23170+23170i 0+32767i 12540+30274i 23170+23170i 30274+12540i]'}  ClassIndex=1  ClassCtorIndex=1  ClassTabVisible=on  ClassTemplateParamsVisible=on  ClassCtorDeclVisible=on  ClassCtorParamsVisible=on  FunctionTabVisible=on  FunctionDecl=|  PortAttrs={ 'input', 'sig0_i', 'input_stream< TT_DATA > * restrict', '', '', '', ''; 'input', 'sig1_i', 'input_stream< TT_DATA > * restrict', '', '', '', ''; 'input', 'acc_i', 'input_stream< TT_ACC > * restrict', '', '', '', ''; 'output', 'sig0_o', 'output_stream< TT_DATA > * restrict', '', '', '', '4*N'; 'output', 'sig1_o', 'output_stream< TT_DATA > * restrict', '', '', '', '4*N' }  PortAttrsEnables={'off', 'off', 'off', 'off', 'off', 'off', 'off';'off', 'off', 'off', 'off', 'off', 'off', 'off';'off', 'off', 'off', 'off', 'off', 'off', 'off';'off', 'off', 'off', 'off', 'off', 'off', 'on';'off', 'off', 'off', 'off', 'off', 'off', 'on'}  SampleTime=-1  ClassDeclTypeOptions=C[1 1]@t107@template < typename TT_DATA, typename TT_COEFF, typename TT_ACC, unsigned int NSAMP > class dft_1xN_output;  ClassDecl=template < typename TT_DATA, typename TT_COEFF, typename TT_ACC, unsigned int NSAMP > class dft_1xN_output;  ClassTemplateParams={ 'TT_DATA', 'typename', 'cint16'; 'TT_COEFF', 'typename', 'cint16'; 'TT_ACC', 'typename', 'cacc48'; 'NSAMP', 'unsigned int', '4*N' }  ClassTemplateParamsEnables={'off', 'off', 'on';'off', 'off', 'on';'off', 'off', 'on';'off', 'off', 'on'}  ClassCtorDeclTypeOptions=C[1 1]@t76@dft_1xN_output(TT_COEFF ( & coeff0_i ) [ 8 ], TT_COEFF ( & coeff1_i ) [ 8 ])  ClassCtorDecl=dft_1xN_output(TT_COEFF ( & coeff0_i ) [ 8 ], TT_COEFF ( & coeff1_i ) [ 8 ])  ClassCtorParams={ 'coeff0_i', 'TT_COEFF ( &) [ 8 ]', 'twidD0(4,:)'; 'coeff1_i', 'TT_COEFF ( &) [ 8 ]', 'twidD1(4,:)' }  KernelHeaderFile=aie/dft_1xN_widget.h  KernelClassName=dft_1xN_output  KernelFunction=run_output  KernelSourceFile=aie/dft_1xN_widget.cpp  KernelSearchPaths={}  PreProcOptions={}  blockJsonConstraints=[]
      KernelAllAttrs=|
      | s[12;12;9;9;19;14;21;23;21;23;24;21;15;17;12;24;26;26;26;27;28;9;21;23;23;23;24;25;14;19;19;29]@FunctionNameDeclFileNamePortNamesPortTypesPortSerializedTypesPortDirectionsPortWindowSizeEnablesPortWindowMarginEnablesPortBufferSizeEnablesPortBufferMarginEnablesPortSynchronicityEnablesPortSignalSizeEnablesPortBufferSizesPortBufferMarginsFunctionDeclFunctionTemplateSpecKindFunctionTemplateParamNamesFunctionTemplateParamKindsFunctionTemplateParamTypesFunctionTemplateParamValuesFunctionTemplateParamEnablesClassDeclClassTemplateSpecKindClassTemplateParamNamesClassTemplateParamKindsClassTemplateParamTypesClassTemplateParamValuesClassTemplateParamEnablesClassCtorDeclsClassCtorParamNamesClassCtorParamTypesClassCtorParamSerializedTypes[1 1]@C[32 1]@t10@run_outputt22@../../dft_1xN_widget.hC[5 1]@t6@sig0_it6@sig1_it5@acc_it6@sig0_ot6@sig1_oC[5 1]@t34@input_stream< TT_DATA > * restrictt34@input_stream< TT_DATA > * restrictt33@input_stream< TT_ACC > * restrictt35@output_stream< TT_DATA > * restrictt35@output_stream< TT_DATA > * restrictC[5 1]@t38@{Q2{P{Tinput_stream{1{t{ETT_DATA}}}}}}t38@{Q2{P{Tinput_stream{1{t{ETT_DATA}}}}}}t37@{Q2{P{Tinput_stream{1{t{ETT_ACC}}}}}}t39@{Q2{P{Toutput_stream{1{t{ETT_DATA}}}}}}t39@{Q2{P{Toutput_stream{1{t{ETT_DATA}}}}}}C[5 1]@t5@inputt5@inputt5@inputt6@outputt6@outputC[5 1]@l0@l0@l0@l0@l0@C[5 1]@l0@l0@l0@l0@l0@C[5 1]@l0@l0@l0@l0@l0@C[5 1]@l0@l0@l0@l0@l0@C[5 1]@l0@l0@l0@l0@l0@C[5 1]@l0@l0@l0@l1@l1@C[5 1]@nnnnnC[5 1]@nnnnnt334@template < typename TT_DATA, typename TT_COEFF, typename TT_ACC, unsigned int NSAMP > 
      | void dft_1xN_output::
      | run_output(input_stream< TT_DATA > * restrict sig0_i, input_stream< TT_DATA > * restrict sig1_i, input_stream< TT_ACC > * restrict acc_i, output_stream< TT_DATA > * restrict sig0_o, output_stream< TT_DATA > * restrict sig1_o)t4@nonee[0 1]@e[0 1]@e[0 1]@e[0 1]@e[0 1]@t107@template < typename TT_DATA, typename TT_COEFF, typename TT_ACC, unsigned int NSAMP > class dft_1xN_output;t8@implicitC[4 1]@t7@TT_DATAt8@TT_COEFFt6@TT_ACCt5@NSAMPC[4 1]@t4@typet4@typet4@typet7@nontypeC[4 1]@t8@typenamet8@typenamet8@typenamet12@unsigned intC[4 1]@nnnnC[4 1]@l1@l1@l1@l1@C[1 1]@t76@dft_1xN_output(TT_COEFF ( & coeff0_i ) [ 8 ], TT_COEFF ( & coeff1_i ) [ 8 ])C[1 1]@C[2 1]@t8@coeff0_it8@coeff1_iC[1 1]@C[2 1]@t19@TT_COEFF ( &) [ 8 ]t19@TT_COEFF ( &) [ 8 ]C[1 1]@C[2 1]@t18@{R{C{ETT_COEFF}8}}t18@{R{C{ETT_COEFF}8}}
      FunctionDecl=|
      | template < typename TT_DATA, typename TT_COEFF, typename TT_ACC, unsigned int NSAMP > 
      | void dft_1xN_output::
      | run_output(input_stream< TT_DATA > * restrict sig0_i, input_stream< TT_DATA > * restrict sig1_i, input_stream< TT_ACC > * restrict acc_i, output_stream< TT_DATA > * restrict sig0_o, output_stream< TT_DATA > * restrict sig1_o)
  u0 : Outport
  u1 : Outport  Port=2
  u2 : Outport  Port=3
  u3 : Outport  Port=4
  u4 : Outport  Port=5
  u5 : Outport  Port=6
  u6 : Outport  Port=7
  u7 : Outport  Port=8
  wires:
  run_output3/2 -> u7/1
  y7/1 -> run_output/2, run_output1/2, run_output2/2, run_output3/2
  run_middle6/1 -> run_middle7/3
  y6/1 -> run_output3/1, run_output/1, run_output1/1, run_output2/1
  run_output/1 -> u0/1
  run_middle5/1 -> run_output2/3
  run_output/2 -> u1/1
  run_output1/2 -> u3/1
  y5/1 -> run_middle7/2, run_middle5/2, run_middle3/2, run_middle1/2
  y3/1 -> run_middle6/2, run_middle4/2, run_middle2/2, run_middle/2
  y2/1 -> run_middle6/1, run_middle4/1, run_middle2/1, run_middle/1
  y0/1 -> run_input2/1, run_input3/1, run_input1/1, run_input/1
  run_output2/2 -> u5/1
  run_output2/1 -> u4/1
  run_middle3/1 -> run_output1/3
  run_input1/1 -> run_middle2/3
  run_middle2/1 -> run_middle3/3
  run_output3/1 -> u6/1
  y1/1 -> run_input3/2, run_input2/2, run_input1/2, run_input/2
  run_middle4/1 -> run_middle5/3
  run_middle7/1 -> run_output3/3
  run_middle/1 -> run_middle1/3
  run_input/1 -> run_middle/3
  y4/1 -> run_middle7/1, run_middle5/1, run_middle3/1, run_middle1/1
  run_output1/1 -> u2/1
  run_input2/1 -> run_middle4/3
  run_input3/1 -> run_middle6/3
  run_middle1/1 -> run_output/3
